simulink model "TIM_5_1_2"  (R2022b)
(part 2 of 4)

  Nex_1 (3) : M-S-Function  FunctionName=cisia_msfun  Parameters=Parameter1, Parameter2, Parameter3, resources, Parameter10, codeupdate, step_received, step_computed, dynamic_computed, step_sended, id_entity, id_project, id_type, name_type, color  mask(S-function:msfcn_unit_delay){Parameter1='Nex_1', Parameter2=1, Parameter3='ORO', resources=*** INPUT RESOURCES *** NUM_INPUTS 5 TLC_CONN (20) TLC_SERVICE (20) CYBER_FAULT (10) POWER (1) ROOM_QoS (1)  *** STATE VARIABLES *** NUM_VARIABLES 17 Operative_Level(NUMERIC)(1)(1) TLC_services(NUMERIC_ARRAY)(20)(0  0  0  0  0  0  0  0  0  0  0  0  0  0  0  0  0  0  0  0) Connection(NUMERIC_ARRAY)(20)(0  0  0  0  0  0  0  0  0  0  0  0  0  0  0  0  0  0  0  0) Dos_attack(NUMERIC)(1)(0) MITM_attack(NUMERIC)(1)(0) Virus_Attack(NUMERIC)(1)(0) Port_Scan_Attack(NUMERIC)(1)(0) Cyber_Fault(NUMERIC_ARRAY)(10)(0  0  0  0  0  0  0  0  0  0) BGP_hijacking(NUMERIC)(1)(0) Mechanical_Fault(NUMERIC)(1)(0) Conn_Fault(NUMERIC)(1)(0) BotNet_Attack(NUMERIC)(1)(0) Data_Corruption(NUMERIC)(1)(0) SW_Change(NUMERIC)(1)(0) Config_Change(NUMERIC)(1)(0) Port_Saturation(NUMERIC)(1)(0) TLC_revoke(NUMERIC_ARRAY)(20)(0  0  0  0  0  0  0  0  0  0  0  0  0  0  0  0  0  0  0  0)  *** OUTPUT RESOURCES *** NUM_OUTPUTS 4 TLC_CONN (20) TLC_SERVICE (20) CYBER_FAULT (10) SWITCHING_QoS (1), Parameter10=off, codeupdate=off, step_received=Connection=max(Connection_init,TLC_CONN);  TLC_services=max(TLC_services_init,TLC_SERVICE); TLC_services=mod(TLC_services,10); TLC_revoke=floor(TLC_SERVICE/10);  Cyber_Fault=max(CYBER_FAULT, transpose([Dos_attack   MITM_attack Virus_Attack Port_Scan_Attack  BGP_hijacking BotNet_Attack Data_Corruption SW_Change Config_Change Port_Saturation]));  Conn_Fault=max([Dos_attack  Mechanical_Fault  1-POWER 1-ROOM_QoS] );  Operative_Level=(1-Conn_Fault)*max(max(TLC_services),0.5)*(1-0.5*max(Cyber_Fault));, step_computed=, dynamic_computed=, step_sended=TLC_CONN=Connection*(1-Conn_Fault); TLC_SERVICE=TLC_services*(1-Conn_Fault)+10*TLC_revoke;  Cyber_Transmitted=min(Cyber_Fault, transpose([0 0 1 0 1 1 0 0 0 1])); CYBER_FAULT=Cyber_Transmitted*(1-Conn_Fault);   SWITCHING_QoS=Operative_Level;, id_entity=3, id_project=38, id_type=2, name_type=Nexus93180Switch, color=#0072BD}
      mask prompts: Parameter1 "entity name"; Parameter2 "sampling time"; Parameter3 "project"; resources "input resources and state variables"; Parameter10 "Bring state variables to output"; codeupdate "update code from mask"
      mask help: This is a level-2 MATLAB file S-function which demonstrates CISIA entity
      mask DialogControl Container1 Prompt: All parameters
      mask Display: image('Icons/Nexus93180Switch.png')
  Nex_2 (4) : M-S-Function  FunctionName=cisia_msfun  Parameters=Parameter1, Parameter2, Parameter3, resources, Parameter10, codeupdate, step_received, step_computed, dynamic_computed, step_sended, id_entity, id_project, id_type, name_type, color  mask(S-function:msfcn_unit_delay){Parameter1='Nex_2', Parameter2=1, Parameter3='ORO', resources=*** INPUT RESOURCES *** NUM_INPUTS 5 TLC_CONN (20) TLC_SERVICE (20) CYBER_FAULT (10) POWER (1) ROOM_QoS (1)  *** STATE VARIABLES *** NUM_VARIABLES 17 Operative_Level(NUMERIC)(1)(1) TLC_services(NUMERIC_ARRAY)(20)(0  0  0  0  0  0  0  0  0  0  0  0  0  0  0  0  0  0  0  0) Connection(NUMERIC_ARRAY)(20)(0  0  0  0  0  0  0  0  0  0  0  0  0  0  0  0  0  0  0  0) Dos_attack(NUMERIC)(1)(0) MITM_attack(NUMERIC)(1)(0) Virus_Attack(NUMERIC)(1)(0) Port_Scan_Attack(NUMERIC)(1)(0) Cyber_Fault(NUMERIC_ARRAY)(10)(0  0  0  0  0  0  0  0  0  0) BGP_hijacking(NUMERIC)(1)(0) Mechanical_Fault(NUMERIC)(1)(0) Conn_Fault(NUMERIC)(1)(0) BotNet_Attack(NUMERIC)(1)(0) Data_Corruption(NUMERIC)(1)(0) SW_Change(NUMERIC)(1)(0) Config_Change(NUMERIC)(1)(0) Port_Saturation(NUMERIC)(1)(0) TLC_revoke(NUMERIC_ARRAY)(20)(0  0  0  0  0  0  0  0  0  0  0  0  0  0  0  0  0  0  0  0)  *** OUTPUT RESOURCES *** NUM_OUTPUTS 4 TLC_CONN (20) TLC_SERVICE (20) CYBER_FAULT (10) SWITCHING_QoS (1), Parameter10=off, codeupdate=off, step_received=Connection=max(Connection_init,TLC_CONN);  TLC_services=max(TLC_services_init,TLC_SERVICE); TLC_services=mod(TLC_services,10); TLC_revoke=floor(TLC_SERVICE/10);  Cyber_Fault=max(CYBER_FAULT, transpose([Dos_attack   MITM_attack Virus_Attack Port_Scan_Attack  BGP_hijacking BotNet_Attack Data_Corruption SW_Change Config_Change Port_Saturation]));  Conn_Fault=max([Dos_attack  Mechanical_Fault  1-POWER 1-ROOM_QoS] );  Operative_Level=(1-Conn_Fault)*max(max(TLC_services),0.5)*(1-0.5*max(Cyber_Fault));, step_computed=, dynamic_computed=, step_sended=TLC_CONN=Connection*(1-Conn_Fault); TLC_SERVICE=TLC_services*(1-Conn_Fault)+10*TLC_revoke;  Cyber_Transmitted=min(Cyber_Fault, transpose([0 0 1 0 1 1 0 0 0 1])); CYBER_FAULT=Cyber_Transmitted*(1-Conn_Fault);   SWITCHING_QoS=Operative_Level;, id_entity=4, id_project=38, id_type=2, name_type=Nexus93180Switch, color=#0072BD}
      mask prompts: Parameter1 "entity name"; Parameter2 "sampling time"; Parameter3 "project"; resources "input resources and state variables"; Parameter10 "Bring state variables to output"; codeupdate "update code from mask"
      mask help: This is a level-2 MATLAB file S-function which demonstrates CISIA entity
      mask DialogControl Container1 Prompt: All parameters
      mask Display: image('Icons/Nexus93180Switch.png')
  ONU_3 (282) : M-S-Function  FunctionName=cisia_msfun  Parameters=Parameter1, Parameter2, Parameter3, resources, Parameter10, codeupdate, step_received, step_computed, dynamic_computed, step_sended, id_entity, id_project, id_type, name_type, color  mask(S-function:msfcn_unit_delay){Parameter1='ONU_3', Parameter2=1, Parameter3='ORO', resources=*** INPUT RESOURCES *** NUM_INPUTS 4 TLC_SERVICE (20) CYBER_FAULT (10) POWER (1) NGPON_CONN (20)  *** STATE VARIABLES *** NUM_VARIABLES 22 Operative_Level(NUMERIC)(1)(1) TLC_services(NUMERIC_ARRAY)(20)(0  0  0  0  0  0  0  0  0  0  0  0  0  0  0  0  0  0  0  0) Connection(NUMERIC_ARRAY)(20)(0  0  0  0  0  0  0  0  0  0  0  0  0  0  0  0  0  0  0  0) Dos_attack(NUMERIC)(1)(0) MITM_attack(NUMERIC)(1)(0) Virus_Attack(NUMERIC)(1)(0) Port_Scan_Attack(NUMERIC)(1)(0) Cyber_Fault(NUMERIC_ARRAY)(10)(0  0  0  0  0  0  0  0  0  0) MyConn(NUMERIC_ARRAY)(20)(0  0  0  0  0  0  0  0  0  0  0  0  0  0  0  0  0  0  0  0) BGP_hijacking(NUMERIC)(1)(0) Mechanical_Fault(NUMERIC)(1)(0) Conn_Fault(NUMERIC)(1)(0) Consumed_Services(NUMERIC_ARRAY)(20)(0  0  0  0  0  0  0  0  0  0  0  0  0  0  0  0  0  0  0  0) Service_Fault(NUMERIC)(1)(0) Redundancy_Fault(NUMERIC)(1)(0) BotNet_Attack(NUMERIC)(1)(0) Data_Corruption(NUMERIC)(1)(0) SW_Change(NUMERIC)(1)(0) Config_Change(NUMERIC)(1)(0) Port_Saturation(NUMERIC)(1)(0) My_Service(NUMERIC)(1)(0) TLC_revoke(NUMERIC_ARRAY)(20)(0  0  0  0  0  0  0  0  0  0  0  0  0  0  0  0  0  0  0  0)  *** OUTPUT RESOURCES *** NUM_OUTPUTS 3 TLC_SERVICE (20) CYBER_FAULT (10) NGPON_CONN (20), Parameter10=off, codeupdate=off, step_received=Connection=max(Connection_init,NGPON_CONN); TLC_services=max(TLC_services_init,TLC_SERVICE); TLC_services=mod(TLC_services,10); TLC_revoke=floor(TLC_SERVICE/10);  Cyber_Fault=max(CYBER_FAULT, transpose([Dos_attack   MITM_attack Virus_Attack Port_Scan_Attack  BGP_hijacking BotNet_Attack Data_Corruption SW_Change Config_Change Port_Saturation]));  Conn_Fault=max([Dos_attack  Mechanical_Fault  1-POWER] );  Service_Fault=max(abs(Consumed_Services.*TLC_services-Consumed_Services)); Redundancy_Fault=max(abs(Consumed_Services.*NGPON_CONN-Consumed_Services));  Operative_Level=(1-Conn_Fault)*(1-0.5*max(Cyber_Fault))*(1-Service_Fault)*max(max(NGPON_CONN),0.5);  %Operative_Level=(1-Conn_Fault)*max(max(TLC_services),0.5)*((2*(1-Service_Fault)+(1-Redundancy_Fault))/3); % Il servizio utilizzato %My_Service=max([(1-Service_Fault) (1-Redundancy_Fault)/2]); %Operative_Level=(1-Conn_Fault);, step_computed=, dynamic_computed=, step_sended=TLC_SERVICE=TLC_services*(1-Conn_Fault)+10*TLC_revoke; NGPON_CONN=Connection*(1-Conn_Fault);  Cyber_Transmitted=min(Cyber_Fault, transpose([0 0 1 0 1 1 0 0 0 1])); CYBER_FAULT=Cyber_Transmitted*(1-Conn_Fault);, id_entity=282, id_project=38, id_type=12, name_type=ONU, color=#90DB5A}
      mask prompts: Parameter1 "entity name"; Parameter2 "sampling time"; Parameter3 "project"; resources "input resources and state variables"; Parameter10 "Bring state variables to output"; codeupdate "update code from mask"
      mask help: This is a level-2 MATLAB file S-function which demonstrates CISIA entity
      mask DialogControl Container1 Prompt: All parameters
      mask Display: disp('ONU')
  Operating_1 (177) : M-S-Function  FunctionName=cisia_msfun  Parameters=Parameter1, Parameter2, Parameter3, resources, Parameter10, codeupdate, step_received, step_computed, dynamic_computed, step_sended, id_entity, id_project, id_type, name_type, color  mask(S-function:msfcn_unit_delay){Parameter1='Operating_1', Parameter2=1, Parameter3='ORO', resources=*** INPUT RESOURCES *** NUM_INPUTS 8 TLC_CONN (20) TLC_SERVICE (20) CYBER_FAULT (10) POWER (1) WATER (1) AIR (1) MOBILE_QoS (1) OXYGEN (1)  *** STATE VARIABLES *** NUM_VARIABLES 17 Operative_Level(NUMERIC)(1)(1) TLC_services(NUMERIC_ARRAY)(20)(0  0  0  0  0  0  0  0  0  0  0  0  0  0  0  0  0  0  0  0) Connection(NUMERIC_ARRAY)(20)(0  0  0  0  0  0  0  0  0  0  0  0  0  0  0  0  0  0  0  0) Mechanical_Fault(NUMERIC)(1)(0) Power_Fault(NUMERIC)(1)(0) Fire_Fault(NUMERIC)(1)(0) Conn_Fault(NUMERIC)(1)(0) Consumed_Services(NUMERIC_ARRAY)(20)(0  0  0  0  1  0  0  0  1  0  0  0  0  0  0  0  0  0  0  0) Service_Fault(NUMERIC)(1)(0) Redundancy_Fault(NUMERIC)(1)(0) Water_Fault(NUMERIC)(1)(0) Air_Fault(NUMERIC)(1)(0) Physical_Fault(NUMERIC)(1)(0) TLC_revoke(NUMERIC_ARRAY)(20)(0  0  0  0  0  0  0  0  0  0  0  0  0  0  0  0  0  0  0  0) Alternative_Services(NUMERIC_ARRAY)(20)(0  0  0  0  0  0  0  0  0  0  0  0  0  0  0  0  0  0  0  0) Alt_Serv_Fault(NUMERIC)(1)(0) Alt_Rout_Fault(NUMERIC)(1)(0)  *** OUTPUT RESOURCES *** NUM_OUTPUTS 3 MEDICAL_ROOM_QoS (1) ALT_ROUTING (1) ALT_SERVICES (1), Parameter10=off, codeupdate=off, step_received=Connection=max(Connection_init,TLC_CONN); TLC_services=max(TLC_services_init,TLC_SERVICE); TLC_services=mod(TLC_services,10); TLC_revoke=floor(TLC_SERVICE/10);  Conn_Fault=max([Power_Fault 1-POWER 1-MOBILE_QoS]);  Water_Fault=1-WATER; Air_Fault=1-AIR; Physical_Fault=max([Water_Fault Air_Fault 1-OXYGEN]);  Alt_Serv_Fault=max(abs(Alternative_Services.*TLC_CONN-Alternative_Services));  Alt_Rout_Fault=max(abs(Consumed_Services.*TLC_CONN-Consumed_Services));   Service_Fault=max(abs(Consumed_Services.*TLC_services-Consumed_Services)); Redundancy_Fault=max(abs(Consumed_Services.*TLC_CONN-Consumed_Services));  Operative_Level=(1-Conn_Fault)*(1-0.5*Physical_Fault)*(1-0.5*Service_Fault);, step_computed=, dynamic_computed=, step_sended=MEDICAL_ROOM_QoS=Operative_Level;  ALT_SERVICES=1-Alt_Serv_Fault; ALT_ROUTING=1-Alt_Rout_Fault;, id_entity=177, id_project=38, id_type=25, name_type=Medical_Room, color=#00FFFF}
      mask prompts: Parameter1 "entity name"; Parameter2 "sampling time"; Parameter3 "project"; resources "input resources and state variables"; Parameter10 "Bring state variables to output"; codeupdate "update code from mask"
      mask help: This is a level-2 MATLAB file S-function which demonstrates CISIA entity
      mask DialogControl Container1 Prompt: All parameters
      mask Display: disp('Medical_Room')
  Operating_2 (178) : M-S-Function  FunctionName=cisia_msfun  Parameters=Parameter1, Parameter2, Parameter3, resources, Parameter10, codeupdate, step_received, step_computed, dynamic_computed, step_sended, id_entity, id_project, id_type, name_type, color  mask(S-function:msfcn_unit_delay){Parameter1='Operating_2', Parameter2=1, Parameter3='ORO', resources=*** INPUT RESOURCES *** NUM_INPUTS 8 TLC_CONN (20) TLC_SERVICE (20) CYBER_FAULT (10) POWER (1) WATER (1) AIR (1) MOBILE_QoS (1) OXYGEN (1)  *** STATE VARIABLES *** NUM_VARIABLES 17 Operative_Level(NUMERIC)(1)(1) TLC_services(NUMERIC_ARRAY)(20)(0  0  0  0  0  0  0  0  0  0  0  0  0  0  0  0  0  0  0  0) Connection(NUMERIC_ARRAY)(20)(0  0  0  0  0  0  0  0  0  0  0  0  0  0  0  0  0  0  0  0) Mechanical_Fault(NUMERIC)(1)(0) Power_Fault(NUMERIC)(1)(0) Fire_Fault(NUMERIC)(1)(0) Conn_Fault(NUMERIC)(1)(0) Consumed_Services(NUMERIC_ARRAY)(20)(0  0  0  0  1  0  0  0  1  0  0  0  0  0  0  0  0  0  0  0) Service_Fault(NUMERIC)(1)(0) Redundancy_Fault(NUMERIC)(1)(0) Water_Fault(NUMERIC)(1)(0) Air_Fault(NUMERIC)(1)(0) Physical_Fault(NUMERIC)(1)(0) TLC_revoke(NUMERIC_ARRAY)(20)(0  0  0  0  0  0  0  0  0  0  0  0  0  0  0  0  0  0  0  0) Alternative_Services(NUMERIC_ARRAY)(20)(0  0  0  0  0  0  0  0  0  0  0  0  0  0  0  0  0  0  0  0) Alt_Serv_Fault(NUMERIC)(1)(0) Alt_Rout_Fault(NUMERIC)(1)(0)  *** OUTPUT RESOURCES *** NUM_OUTPUTS 3 MEDICAL_ROOM_QoS (1) ALT_ROUTING (1) ALT_SERVICES (1), Parameter10=off, codeupdate=off, step_received=Connection=max(Connection_init,TLC_CONN); TLC_services=max(TLC_services_init,TLC_SERVICE); TLC_services=mod(TLC_services,10); TLC_revoke=floor(TLC_SERVICE/10);  Conn_Fault=max([Power_Fault 1-POWER 1-MOBILE_QoS]);  Water_Fault=1-WATER; Air_Fault=1-AIR; Physical_Fault=max([Water_Fault Air_Fault 1-OXYGEN]);  Alt_Serv_Fault=max(abs(Alternative_Services.*TLC_CONN-Alternative_Services));  Alt_Rout_Fault=max(abs(Consumed_Services.*TLC_CONN-Consumed_Services));   Service_Fault=max(abs(Consumed_Services.*TLC_services-Consumed_Services)); Redundancy_Fault=max(abs(Consumed_Services.*TLC_CONN-Consumed_Services));  Operative_Level=(1-Conn_Fault)*(1-0.5*Physical_Fault)*(1-0.5*Service_Fault);, step_computed=, dynamic_computed=, step_sended=MEDICAL_ROOM_QoS=Operative_Level;  ALT_SERVICES=1-Alt_Serv_Fault; ALT_ROUTING=1-Alt_Rout_Fault;, id_entity=178, id_project=38, id_type=25, name_type=Medical_Room, color=#00FFFF}
      mask prompts: Parameter1 "entity name"; Parameter2 "sampling time"; Parameter3 "project"; resources "input resources and state variables"; Parameter10 "Bring state variables to output"; codeupdate "update code from mask"
      mask help: This is a level-2 MATLAB file S-function which demonstrates CISIA entity
      mask DialogControl Container1 Prompt: All parameters
      mask Display: disp('Medical_Room')
  Oxygen_Duct_1 (263) : M-S-Function  FunctionName=cisia_msfun  Parameters=Parameter1, Parameter2, Parameter3, resources, Parameter10, codeupdate, step_received, step_computed, dynamic_computed, step_sended, id_entity, id_project, id_type, name_type, color  mask(S-function:msfcn_unit_delay){Parameter1='Oxygen_Duct_1', Parameter2=1, Parameter3='ORO', resources=*** INPUT RESOURCES *** NUM_INPUTS 1 OXYGEN (1)  *** STATE VARIABLES *** NUM_VARIABLES 2 Operative_Level(NUMERIC)(1)(1) Mechanical_Fault(NUMERIC)(1)(0)  *** OUTPUT RESOURCES *** NUM_OUTPUTS 1 OXYGEN (1), Parameter10=off, codeupdate=off, step_received=Operative_Level=(1-Mechanical_Fault)*(1-0.5*(1-OXYGEN));, step_computed=, dynamic_computed=, step_sended=OXYGEN=Operative_Level;, id_entity=263, id_project=38, id_type=57, name_type=OXYGEN_Duct, color=#E85151}
      mask prompts: Parameter1 "entity name"; Parameter2 "sampling time"; Parameter3 "project"; resources "input resources and state variables"; Parameter10 "Bring state variables to output"; codeupdate "update code from mask"
      mask help: This is a level-2 MATLAB file S-function which demonstrates CISIA entity
      mask DialogControl Container1 Prompt: All parameters
      mask Display: disp('OXYGEN_Duct')
  Oxygen_Duct_2 (264) : M-S-Function  FunctionName=cisia_msfun  Parameters=Parameter1, Parameter2, Parameter3, resources, Parameter10, codeupdate, step_received, step_computed, dynamic_computed, step_sended, id_entity, id_project, id_type, name_type, color  mask(S-function:msfcn_unit_delay){Parameter1='Oxygen_Duct_2', Parameter2=1, Parameter3='ORO', resources=*** INPUT RESOURCES *** NUM_INPUTS 1 OXYGEN (1)  *** STATE VARIABLES *** NUM_VARIABLES 2 Operative_Level(NUMERIC)(1)(1) Mechanical_Fault(NUMERIC)(1)(0)  *** OUTPUT RESOURCES *** NUM_OUTPUTS 1 OXYGEN (1), Parameter10=off, codeupdate=off, step_received=Operative_Level=(1-Mechanical_Fault)*(1-0.5*(1-OXYGEN));, step_computed=, dynamic_computed=, step_sended=OXYGEN=Operative_Level;, id_entity=264, id_project=38, id_type=57, name_type=OXYGEN_Duct, color=#E85151}
      mask prompts: Parameter1 "entity name"; Parameter2 "sampling time"; Parameter3 "project"; resources "input resources and state variables"; Parameter10 "Bring state variables to output"; codeupdate "update code from mask"
      mask help: This is a level-2 MATLAB file S-function which demonstrates CISIA entity
      mask DialogControl Container1 Prompt: All parameters
      mask Display: disp('OXYGEN_Duct')
  Oxygen_Duct_3 (265) : M-S-Function  FunctionName=cisia_msfun  Parameters=Parameter1, Parameter2, Parameter3, resources, Parameter10, codeupdate, step_received, step_computed, dynamic_computed, step_sended, id_entity, id_project, id_type, name_type, color  mask(S-function:msfcn_unit_delay){Parameter1='Oxygen_Duct_3', Parameter2=1, Parameter3='ORO', resources=*** INPUT RESOURCES *** NUM_INPUTS 1 OXYGEN (1)  *** STATE VARIABLES *** NUM_VARIABLES 2 Operative_Level(NUMERIC)(1)(1) Mechanical_Fault(NUMERIC)(1)(0)  *** OUTPUT RESOURCES *** NUM_OUTPUTS 1 OXYGEN (1), Parameter10=off, codeupdate=off, step_received=Operative_Level=(1-Mechanical_Fault)*(1-0.5*(1-OXYGEN));, step_computed=, dynamic_computed=, step_sended=OXYGEN=Operative_Level;, id_entity=265, id_project=38, id_type=57, name_type=OXYGEN_Duct, color=#E85151}
      mask prompts: Parameter1 "entity name"; Parameter2 "sampling time"; Parameter3 "project"; resources "input resources and state variables"; Parameter10 "Bring state variables to output"; codeupdate "update code from mask"
      mask help: This is a level-2 MATLAB file S-function which demonstrates CISIA entity
      mask DialogControl Container1 Prompt: All parameters
      mask Display: disp('OXYGEN_Duct')
  Oxygen_Duct_4 (266) : M-S-Function  FunctionName=cisia_msfun  Parameters=Parameter1, Parameter2, Parameter3, resources, Parameter10, codeupdate, step_received, step_computed, dynamic_computed, step_sended, id_entity, id_project, id_type, name_type, color  mask(S-function:msfcn_unit_delay){Parameter1='Oxygen_Duct_4', Parameter2=1, Parameter3='ORO', resources=*** INPUT RESOURCES *** NUM_INPUTS 1 OXYGEN (1)  *** STATE VARIABLES *** NUM_VARIABLES 2 Operative_Level(NUMERIC)(1)(1) Mechanical_Fault(NUMERIC)(1)(0)  *** OUTPUT RESOURCES *** NUM_OUTPUTS 1 OXYGEN (1), Parameter10=off, codeupdate=off, step_received=Operative_Level=(1-Mechanical_Fault)*(1-0.5*(1-OXYGEN));, step_computed=, dynamic_computed=, step_sended=OXYGEN=Operative_Level;, id_entity=266, id_project=38, id_type=57, name_type=OXYGEN_Duct, color=#E85151}
      mask prompts: Parameter1 "entity name"; Parameter2 "sampling time"; Parameter3 "project"; resources "input resources and state variables"; Parameter10 "Bring state variables to output"; codeupdate "update code from mask"
      mask help: This is a level-2 MATLAB file S-function which demonstrates CISIA entity
      mask DialogControl Container1 Prompt: All parameters
      mask Display: disp('OXYGEN_Duct')
  Oxygen_Duct_5 (267) : M-S-Function  FunctionName=cisia_msfun  Parameters=Parameter1, Parameter2, Parameter3, resources, Parameter10, codeupdate, step_received, step_computed, dynamic_computed, step_sended, id_entity, id_project, id_type, name_type, color  mask(S-function:msfcn_unit_delay){Parameter1='Oxygen_Duct_5', Parameter2=1, Parameter3='ORO', resources=*** INPUT RESOURCES *** NUM_INPUTS 1 OXYGEN (1)  *** STATE VARIABLES *** NUM_VARIABLES 2 Operative_Level(NUMERIC)(1)(1) Mechanical_Fault(NUMERIC)(1)(0)  *** OUTPUT RESOURCES *** NUM_OUTPUTS 1 OXYGEN (1), Parameter10=off, codeupdate=off, step_received=Operative_Level=(1-Mechanical_Fault)*(1-0.5*(1-OXYGEN));, step_computed=, dynamic_computed=, step_sended=OXYGEN=Operative_Level;, id_entity=267, id_project=38, id_type=57, name_type=OXYGEN_Duct, color=#E85151}
      mask prompts: Parameter1 "entity name"; Parameter2 "sampling time"; Parameter3 "project"; resources "input resources and state variables"; Parameter10 "Bring state variables to output"; codeupdate "update code from mask"
      mask help: This is a level-2 MATLAB file S-function which demonstrates CISIA entity
      mask DialogControl Container1 Prompt: All parameters
      mask Display: disp('OXYGEN_Duct')
  Oxygen_Duct_6 (268) : M-S-Function  FunctionName=cisia_msfun  Parameters=Parameter1, Parameter2, Parameter3, resources, Parameter10, codeupdate, step_received, step_computed, dynamic_computed, step_sended, id_entity, id_project, id_type, name_type, color  mask(S-function:msfcn_unit_delay){Parameter1='Oxygen_Duct_6', Parameter2=1, Parameter3='ORO', resources=*** INPUT RESOURCES *** NUM_INPUTS 1 OXYGEN (1)  *** STATE VARIABLES *** NUM_VARIABLES 2 Operative_Level(NUMERIC)(1)(1) Mechanical_Fault(NUMERIC)(1)(0)  *** OUTPUT RESOURCES *** NUM_OUTPUTS 1 OXYGEN (1), Parameter10=off, codeupdate=off, step_received=Operative_Level=(1-Mechanical_Fault)*(1-0.5*(1-OXYGEN));, step_computed=, dynamic_computed=, step_sended=OXYGEN=Operative_Level;, id_entity=268, id_project=38, id_type=57, name_type=OXYGEN_Duct, color=#E85151}
      mask prompts: Parameter1 "entity name"; Parameter2 "sampling time"; Parameter3 "project"; resources "input resources and state variables"; Parameter10 "Bring state variables to output"; codeupdate "update code from mask"
      mask help: This is a level-2 MATLAB file S-function which demonstrates CISIA entity
      mask DialogControl Container1 Prompt: All parameters
      mask Display: disp('OXYGEN_Duct')
  Oxygen_Duct_7 (269) : M-S-Function  FunctionName=cisia_msfun  Parameters=Parameter1, Parameter2, Parameter3, resources, Parameter10, codeupdate, step_received, step_computed, dynamic_computed, step_sended, id_entity, id_project, id_type, name_type, color  mask(S-function:msfcn_unit_delay){Parameter1='Oxygen_Duct_7', Parameter2=1, Parameter3='ORO', resources=*** INPUT RESOURCES *** NUM_INPUTS 1 OXYGEN (1)  *** STATE VARIABLES *** NUM_VARIABLES 2 Operative_Level(NUMERIC)(1)(1) Mechanical_Fault(NUMERIC)(1)(0)  *** OUTPUT RESOURCES *** NUM_OUTPUTS 1 OXYGEN (1), Parameter10=off, codeupdate=off, step_received=Operative_Level=(1-Mechanical_Fault)*(1-0.5*(1-OXYGEN));, step_computed=, dynamic_computed=, step_sended=OXYGEN=Operative_Level;, id_entity=269, id_project=38, id_type=57, name_type=OXYGEN_Duct, color=#E85151}
      mask prompts: Parameter1 "entity name"; Parameter2 "sampling time"; Parameter3 "project"; resources "input resources and state variables"; Parameter10 "Bring state variables to output"; codeupdate "update code from mask"
      mask help: This is a level-2 MATLAB file S-function which demonstrates CISIA entity
      mask DialogControl Container1 Prompt: All parameters
      mask Display: disp('OXYGEN_Duct')
  Oxygen_Duct_8 (270) : M-S-Function  FunctionName=cisia_msfun  Parameters=Parameter1, Parameter2, Parameter3, resources, Parameter10, codeupdate, step_received, step_computed, dynamic_computed, step_sended, id_entity, id_project, id_type, name_type, color  mask(S-function:msfcn_unit_delay){Parameter1='Oxygen_Duct_8', Parameter2=1, Parameter3='ORO', resources=*** INPUT RESOURCES *** NUM_INPUTS 1 OXYGEN (1)  *** STATE VARIABLES *** NUM_VARIABLES 2 Operative_Level(NUMERIC)(1)(1) Mechanical_Fault(NUMERIC)(1)(0)  *** OUTPUT RESOURCES *** NUM_OUTPUTS 1 OXYGEN (1), Parameter10=off, codeupdate=off, step_received=Operative_Level=(1-Mechanical_Fault)*(1-0.5*(1-OXYGEN));, step_computed=, dynamic_computed=, step_sended=OXYGEN=Operative_Level;, id_entity=270, id_project=38, id_type=57, name_type=OXYGEN_Duct, color=#E85151}
      mask prompts: Parameter1 "entity name"; Parameter2 "sampling time"; Parameter3 "project"; resources "input resources and state variables"; Parameter10 "Bring state variables to output"; codeupdate "update code from mask"
      mask help: This is a level-2 MATLAB file S-function which demonstrates CISIA entity
      mask DialogControl Container1 Prompt: All parameters
      mask Display: disp('OXYGEN_Duct')
  Oxygen_Pump (251) : M-S-Function  FunctionName=cisia_msfun  Parameters=Parameter1, Parameter2, Parameter3, resources, Parameter10, codeupdate, step_received, step_computed, dynamic_computed, step_sended, id_entity, id_project, id_type, name_type, color  mask(S-function:msfcn_unit_delay){Parameter1='Oxygen_Pump', Parameter2=1, Parameter3='ORO', resources=*** INPUT RESOURCES *** NUM_INPUTS 1 POWER (1)  *** STATE VARIABLES *** NUM_VARIABLES 3 Operative_Level(NUMERIC)(1)(1) Mechanical_Fault(NUMERIC)(1)(0) Power_Fault(NUMERIC)(1)(0)  *** OUTPUT RESOURCES *** NUM_OUTPUTS 1 OXYGEN (1), Parameter10=off, codeupdate=off, step_received=Power_Fault=(1-POWER); Operative_Level=(1-Mechanical_Fault)*(1-0.5*Power_Fault);, step_computed=, dynamic_computed=, step_sended=OXYGEN=Operative_Level;, id_entity=251, id_project=38, id_type=56, name_type=OXYGEN_Element, color=#A11326}
      mask prompts: Parameter1 "entity name"; Parameter2 "sampling time"; Parameter3 "project"; resources "input resources and state variables"; Parameter10 "Bring state variables to output"; codeupdate "update code from mask"
      mask help: This is a level-2 MATLAB file S-function which demonstrates CISIA entity
      mask DialogControl Container1 Prompt: All parameters
      mask Display: disp('OXYGEN_Element')
  Pipe_1 (120) : M-S-Function  FunctionName=cisia_msfun  Parameters=Parameter1, Parameter2, Parameter3, resources, Parameter10, codeupdate, step_received, step_computed, dynamic_computed, step_sended, id_entity, id_project, id_type, name_type, color  mask(S-function:msfcn_unit_delay){Parameter1='Pipe_1', Parameter2=1, Parameter3='ORO', resources=*** INPUT RESOURCES *** NUM_INPUTS 1 WATER (1)  *** STATE VARIABLES *** NUM_VARIABLES 3 Operative_Level(NUMERIC)(1)(1) Mechanical_Fault(NUMERIC)(1)(0) Water_Fault(NUMERIC)(1)(0)  *** OUTPUT RESOURCES *** NUM_OUTPUTS 2 WATER (1) PIPE_QoS (1), Parameter10=off, codeupdate=off, step_received=Water_Fault= 1- WATER; Operative_Level=(1-Mechanical_Fault)*(1-0.5*Water_Fault);, step_computed=, dynamic_computed=, step_sended=WATER=Operative_Level; PIPE_QoS=Operative_Level;, id_entity=120, id_project=38, id_type=32, name_type=Pipe, color=#78C6FA}
      mask prompts: Parameter1 "entity name"; Parameter2 "sampling time"; Parameter3 "project"; resources "input resources and state variables"; Parameter10 "Bring state variables to output"; codeupdate "update code from mask"
      mask help: This is a level-2 MATLAB file S-function which demonstrates CISIA entity
      mask DialogControl Container1 Prompt: All parameters
      mask Display: image('Icons/Pipe.png')
  Pipe_Medical1 (128) : M-S-Function  FunctionName=cisia_msfun  Parameters=Parameter1, Parameter2, Parameter3, resources, Parameter10, codeupdate, step_received, step_computed, dynamic_computed, step_sended, id_entity, id_project, id_type, name_type, color  mask(S-function:msfcn_unit_delay){Parameter1='Pipe_Medical1', Parameter2=1, Parameter3='ORO', resources=*** INPUT RESOURCES *** NUM_INPUTS 1 WATER (1)  *** STATE VARIABLES *** NUM_VARIABLES 3 Operative_Level(NUMERIC)(1)(1) Mechanical_Fault(NUMERIC)(1)(0) Water_Fault(NUMERIC)(1)(0)  *** OUTPUT RESOURCES *** NUM_OUTPUTS 2 WATER (1) PIPE_QoS (1), Parameter10=off, codeupdate=off, step_received=Water_Fault= 1- WATER; Operative_Level=(1-Mechanical_Fault)*(1-0.5*Water_Fault);, step_computed=, dynamic_computed=, step_sended=WATER=Operative_Level; PIPE_QoS=Operative_Level;, id_entity=128, id_project=38, id_type=32, name_type=Pipe, color=#78C6FA}
      mask prompts: Parameter1 "entity name"; Parameter2 "sampling time"; Parameter3 "project"; resources "input resources and state variables"; Parameter10 "Bring state variables to output"; codeupdate "update code from mask"
      mask help: This is a level-2 MATLAB file S-function which demonstrates CISIA entity
      mask DialogControl Container1 Prompt: All parameters
      mask Display: image('Icons/Pipe.png')
  Pipe_Medical2 (129) : M-S-Function  FunctionName=cisia_msfun  Parameters=Parameter1, Parameter2, Parameter3, resources, Parameter10, codeupdate, step_received, step_computed, dynamic_computed, step_sended, id_entity, id_project, id_type, name_type, color  mask(S-function:msfcn_unit_delay){Parameter1='Pipe_Medical2', Parameter2=1, Parameter3='ORO', resources=*** INPUT RESOURCES *** NUM_INPUTS 1 WATER (1)  *** STATE VARIABLES *** NUM_VARIABLES 3 Operative_Level(NUMERIC)(1)(1) Mechanical_Fault(NUMERIC)(1)(0) Water_Fault(NUMERIC)(1)(0)  *** OUTPUT RESOURCES *** NUM_OUTPUTS 2 WATER (1) PIPE_QoS (1), Parameter10=off, codeupdate=off, step_received=Water_Fault= 1- WATER; Operative_Level=(1-Mechanical_Fault)*(1-0.5*Water_Fault);, step_computed=, dynamic_computed=, step_sended=WATER=Operative_Level; PIPE_QoS=Operative_Level;, id_entity=129, id_project=38, id_type=32, name_type=Pipe, color=#78C6FA}
      mask prompts: Parameter1 "entity name"; Parameter2 "sampling time"; Parameter3 "project"; resources "input resources and state variables"; Parameter10 "Bring state variables to output"; codeupdate "update code from mask"
      mask help: This is a level-2 MATLAB file S-function which demonstrates CISIA entity
      mask DialogControl Container1 Prompt: All parameters
      mask Display: image('Icons/Pipe.png')
  Pipe_Medical3 (130) : M-S-Function  FunctionName=cisia_msfun  Parameters=Parameter1, Parameter2, Parameter3, resources, Parameter10, codeupdate, step_received, step_computed, dynamic_computed, step_sended, id_entity, id_project, id_type, name_type, color  mask(S-function:msfcn_unit_delay){Parameter1='Pipe_Medical3', Parameter2=1, Parameter3='ORO', resources=*** INPUT RESOURCES *** NUM_INPUTS 1 WATER (1)  *** STATE VARIABLES *** NUM_VARIABLES 3 Operative_Level(NUMERIC)(1)(1) Mechanical_Fault(NUMERIC)(1)(0) Water_Fault(NUMERIC)(1)(0)  *** OUTPUT RESOURCES *** NUM_OUTPUTS 2 WATER (1) PIPE_QoS (1), Parameter10=off, codeupdate=off, step_received=Water_Fault= 1- WATER; Operative_Level=(1-Mechanical_Fault)*(1-0.5*Water_Fault);, step_computed=, dynamic_computed=, step_sended=WATER=Operative_Level; PIPE_QoS=Operative_Level;, id_entity=130, id_project=38, id_type=32, name_type=Pipe, color=#78C6FA}
      mask prompts: Parameter1 "entity name"; Parameter2 "sampling time"; Parameter3 "project"; resources "input resources and state variables"; Parameter10 "Bring state variables to output"; codeupdate "update code from mask"
      mask help: This is a level-2 MATLAB file S-function which demonstrates CISIA entity
      mask DialogControl Container1 Prompt: All parameters
      mask Display: image('Icons/Pipe.png')
  Pipe_Medical4 (131) : M-S-Function  FunctionName=cisia_msfun  Parameters=Parameter1, Parameter2, Parameter3, resources, Parameter10, codeupdate, step_received, step_computed, dynamic_computed, step_sended, id_entity, id_project, id_type, name_type, color  mask(S-function:msfcn_unit_delay){Parameter1='Pipe_Medical4', Parameter2=1, Parameter3='ORO', resources=*** INPUT RESOURCES *** NUM_INPUTS 1 WATER (1)  *** STATE VARIABLES *** NUM_VARIABLES 3 Operative_Level(NUMERIC)(1)(1) Mechanical_Fault(NUMERIC)(1)(0) Water_Fault(NUMERIC)(1)(0)  *** OUTPUT RESOURCES *** NUM_OUTPUTS 2 WATER (1) PIPE_QoS (1), Parameter10=off, codeupdate=off, step_received=Water_Fault= 1- WATER; Operative_Level=(1-Mechanical_Fault)*(1-0.5*Water_Fault);, step_computed=, dynamic_computed=, step_sended=WATER=Operative_Level; PIPE_QoS=Operative_Level;, id_entity=131, id_project=38, id_type=32, name_type=Pipe, color=#78C6FA}
      mask prompts: Parameter1 "entity name"; Parameter2 "sampling time"; Parameter3 "project"; resources "input resources and state variables"; Parameter10 "Bring state variables to output"; codeupdate "update code from mask"
      mask help: This is a level-2 MATLAB file S-function which demonstrates CISIA entity
      mask DialogControl Container1 Prompt: All parameters
      mask Display: image('Icons/Pipe.png')
  Pipe_Medical5 (132) : M-S-Function  FunctionName=cisia_msfun  Parameters=Parameter1, Parameter2, Parameter3, resources, Parameter10, codeupdate, step_received, step_computed, dynamic_computed, step_sended, id_entity, id_project, id_type, name_type, color  mask(S-function:msfcn_unit_delay){Parameter1='Pipe_Medical5', Parameter2=1, Parameter3='ORO', resources=*** INPUT RESOURCES *** NUM_INPUTS 1 WATER (1)  *** STATE VARIABLES *** NUM_VARIABLES 3 Operative_Level(NUMERIC)(1)(1) Mechanical_Fault(NUMERIC)(1)(0) Water_Fault(NUMERIC)(1)(0)  *** OUTPUT RESOURCES *** NUM_OUTPUTS 2 WATER (1) PIPE_QoS (1), Parameter10=off, codeupdate=off, step_received=Water_Fault= 1- WATER; Operative_Level=(1-Mechanical_Fault)*(1-0.5*Water_Fault);, step_computed=, dynamic_computed=, step_sended=WATER=Operative_Level; PIPE_QoS=Operative_Level;, id_entity=132, id_project=38, id_type=32, name_type=Pipe, color=#78C6FA}
      mask prompts: Parameter1 "entity name"; Parameter2 "sampling time"; Parameter3 "project"; resources "input resources and state variables"; Parameter10 "Bring state variables to output"; codeupdate "update code from mask"
      mask help: This is a level-2 MATLAB file S-function which demonstrates CISIA entity
      mask DialogControl Container1 Prompt: All parameters
      mask Display: image('Icons/Pipe.png')
  Pipe_Medical6 (133) : M-S-Function  FunctionName=cisia_msfun  Parameters=Parameter1, Parameter2, Parameter3, resources, Parameter10, codeupdate, step_received, step_computed, dynamic_computed, step_sended, id_entity, id_project, id_type, name_type, color  mask(S-function:msfcn_unit_delay){Parameter1='Pipe_Medical6', Parameter2=1, Parameter3='ORO', resources=*** INPUT RESOURCES *** NUM_INPUTS 1 WATER (1)  *** STATE VARIABLES *** NUM_VARIABLES 3 Operative_Level(NUMERIC)(1)(1) Mechanical_Fault(NUMERIC)(1)(0) Water_Fault(NUMERIC)(1)(0)  *** OUTPUT RESOURCES *** NUM_OUTPUTS 2 WATER (1) PIPE_QoS (1), Parameter10=off, codeupdate=off, step_received=Water_Fault= 1- WATER; Operative_Level=(1-Mechanical_Fault)*(1-0.5*Water_Fault);, step_computed=, dynamic_computed=, step_sended=WATER=Operative_Level; PIPE_QoS=Operative_Level;, id_entity=133, id_project=38, id_type=32, name_type=Pipe, color=#78C6FA}
      mask prompts: Parameter1 "entity name"; Parameter2 "sampling time"; Parameter3 "project"; resources "input resources and state variables"; Parameter10 "Bring state variables to output"; codeupdate "update code from mask"
      mask help: This is a level-2 MATLAB file S-function which demonstrates CISIA entity
      mask DialogControl Container1 Prompt: All parameters
      mask Display: image('Icons/Pipe.png')
  Pipe_Oper1 (134) : M-S-Function  FunctionName=cisia_msfun  Parameters=Parameter1, Parameter2, Parameter3, resources, Parameter10, codeupdate, step_received, step_computed, dynamic_computed, step_sended, id_entity, id_project, id_type, name_type, color  mask(S-function:msfcn_unit_delay){Parameter1='Pipe_Oper1', Parameter2=1, Parameter3='ORO', resources=*** INPUT RESOURCES *** NUM_INPUTS 1 WATER (1)  *** STATE VARIABLES *** NUM_VARIABLES 3 Operative_Level(NUMERIC)(1)(1) Mechanical_Fault(NUMERIC)(1)(0) Water_Fault(NUMERIC)(1)(0)  *** OUTPUT RESOURCES *** NUM_OUTPUTS 2 WATER (1) PIPE_QoS (1), Parameter10=off, codeupdate=off, step_received=Water_Fault= 1- WATER; Operative_Level=(1-Mechanical_Fault)*(1-0.5*Water_Fault);, step_computed=, dynamic_computed=, step_sended=WATER=Operative_Level; PIPE_QoS=Operative_Level;, id_entity=134, id_project=38, id_type=32, name_type=Pipe, color=#78C6FA}
      mask prompts: Parameter1 "entity name"; Parameter2 "sampling time"; Parameter3 "project"; resources "input resources and state variables"; Parameter10 "Bring state variables to output"; codeupdate "update code from mask"
      mask help: This is a level-2 MATLAB file S-function which demonstrates CISIA entity
      mask DialogControl Container1 Prompt: All parameters
      mask Display: image('Icons/Pipe.png')
  Pipe_Oper2 (135) : M-S-Function  FunctionName=cisia_msfun  Parameters=Parameter1, Parameter2, Parameter3, resources, Parameter10, codeupdate, step_received, step_computed, dynamic_computed, step_sended, id_entity, id_project, id_type, name_type, color  mask(S-function:msfcn_unit_delay){Parameter1='Pipe_Oper2', Parameter2=1, Parameter3='ORO', resources=*** INPUT RESOURCES *** NUM_INPUTS 1 WATER (1)  *** STATE VARIABLES *** NUM_VARIABLES 3 Operative_Level(NUMERIC)(1)(1) Mechanical_Fault(NUMERIC)(1)(0) Water_Fault(NUMERIC)(1)(0)  *** OUTPUT RESOURCES *** NUM_OUTPUTS 2 WATER (1) PIPE_QoS (1), Parameter10=off, codeupdate=off, step_received=Water_Fault= 1- WATER; Operative_Level=(1-Mechanical_Fault)*(1-0.5*Water_Fault);, step_computed=, dynamic_computed=, step_sended=WATER=Operative_Level; PIPE_QoS=Operative_Level;, id_entity=135, id_project=38, id_type=32, name_type=Pipe, color=#78C6FA}
      mask prompts: Parameter1 "entity name"; Parameter2 "sampling time"; Parameter3 "project"; resources "input resources and state variables"; Parameter10 "Bring state variables to output"; codeupdate "update code from mask"
      mask help: This is a level-2 MATLAB file S-function which demonstrates CISIA entity
      mask DialogControl Container1 Prompt: All parameters
      mask Display: image('Icons/Pipe.png')
  Pipe_Ward (127) : M-S-Function  FunctionName=cisia_msfun  Parameters=Parameter1, Parameter2, Parameter3, resources, Parameter10, codeupdate, step_received, step_computed, dynamic_computed, step_sended, id_entity, id_project, id_type, name_type, color  mask(S-function:msfcn_unit_delay){Parameter1='Pipe_Ward', Parameter2=1, Parameter3='ORO', resources=*** INPUT RESOURCES *** NUM_INPUTS 1 WATER (1)  *** STATE VARIABLES *** NUM_VARIABLES 3 Operative_Level(NUMERIC)(1)(1) Mechanical_Fault(NUMERIC)(1)(0) Water_Fault(NUMERIC)(1)(0)  *** OUTPUT RESOURCES *** NUM_OUTPUTS 2 WATER (1) PIPE_QoS (1), Parameter10=off, codeupdate=off, step_received=Water_Fault= 1- WATER; Operative_Level=(1-Mechanical_Fault)*(1-0.5*Water_Fault);, step_computed=, dynamic_computed=, step_sended=WATER=Operative_Level; PIPE_QoS=Operative_Level;, id_entity=127, id_project=38, id_type=32, name_type=Pipe, color=#78C6FA}
      mask prompts: Parameter1 "entity name"; Parameter2 "sampling time"; Parameter3 "project"; resources "input resources and state variables"; Parameter10 "Bring state variables to output"; codeupdate "update code from mask"
      mask help: This is a level-2 MATLAB file S-function which demonstrates CISIA entity
      mask DialogControl Container1 Prompt: All parameters
      mask Display: image('Icons/Pipe.png')
  PowerGen_1 (46) : M-S-Function  FunctionName=cisia_msfun  Parameters=Parameter1, Parameter2, Parameter3, resources, Parameter10, codeupdate, step_received, step_computed, dynamic_computed, step_sended, id_entity, id_project, id_type, name_type, color  mask(S-function:msfcn_unit_delay){Parameter1='PowerGen_1', Parameter2=1, Parameter3='ORO', resources=*** INPUT RESOURCES *** NUM_INPUTS 0  *** STATE VARIABLES *** NUM_VARIABLES 2 Operative_Level(NUMERIC)(1)(1) Power_Fault(NUMERIC)(1)(0)  *** OUTPUT RESOURCES *** NUM_OUTPUTS 1 POWER (1), Parameter10=off, codeupdate=off, step_received=Operative_Level=1-Power_Fault;, step_computed=, dynamic_computed=, step_sended=POWER=Operative_Level;, id_entity=46, id_project=38, id_type=8, name_type=PowerSource, color=#84BD8C}
      mask prompts: Parameter1 "entity name"; Parameter2 "sampling time"; Parameter3 "project"; resources "input resources and state variables"; Parameter10 "Bring state variables to output"; codeupdate "update code from mask"
      mask help: This is a level-2 MATLAB file S-function which demonstrates CISIA entity
      mask DialogControl Container1 Prompt: All parameters
      mask Display: image('Icons/PowerSource.png')
  PowerGen_10 (293) : M-S-Function  FunctionName=cisia_msfun  Parameters=Parameter1, Parameter2, Parameter3, resources, Parameter10, codeupdate, step_received, step_computed, dynamic_computed, step_sended, id_entity, id_project, id_type, name_type, color  mask(S-function:msfcn_unit_delay){Parameter1='PowerGen_10', Parameter2=1, Parameter3='ORO', resources=*** INPUT RESOURCES *** NUM_INPUTS 0  *** STATE VARIABLES *** NUM_VARIABLES 2 Operative_Level(NUMERIC)(1)(1) Power_Fault(NUMERIC)(1)(0)  *** OUTPUT RESOURCES *** NUM_OUTPUTS 1 POWER (1), Parameter10=off, codeupdate=off, step_received=Operative_Level=1-Power_Fault;, step_computed=, dynamic_computed=, step_sended=POWER=Operative_Level;, id_entity=293, id_project=38, id_type=8, name_type=PowerSource, color=#84BD8C}
      mask prompts: Parameter1 "entity name"; Parameter2 "sampling time"; Parameter3 "project"; resources "input resources and state variables"; Parameter10 "Bring state variables to output"; codeupdate "update code from mask"
      mask help: This is a level-2 MATLAB file S-function which demonstrates CISIA entity
      mask DialogControl Container1 Prompt: All parameters
      mask Display: image('Icons/PowerSource.png')
  PowerGen_2 (47) : M-S-Function  FunctionName=cisia_msfun  Parameters=Parameter1, Parameter2, Parameter3, resources, Parameter10, codeupdate, step_received, step_computed, dynamic_computed, step_sended, id_entity, id_project, id_type, name_type, color  mask(S-function:msfcn_unit_delay){Parameter1='PowerGen_2', Parameter2=1, Parameter3='ORO', resources=*** INPUT RESOURCES *** NUM_INPUTS 0  *** STATE VARIABLES *** NUM_VARIABLES 2 Operative_Level(NUMERIC)(1)(1) Power_Fault(NUMERIC)(1)(0)  *** OUTPUT RESOURCES *** NUM_OUTPUTS 1 POWER (1), Parameter10=off, codeupdate=off, step_received=Operative_Level=1-Power_Fault;, step_computed=, dynamic_computed=, step_sended=POWER=Operative_Level;, id_entity=47, id_project=38, id_type=8, name_type=PowerSource, color=#84BD8C}
      mask prompts: Parameter1 "entity name"; Parameter2 "sampling time"; Parameter3 "project"; resources "input resources and state variables"; Parameter10 "Bring state variables to output"; codeupdate "update code from mask"
      mask help: This is a level-2 MATLAB file S-function which demonstrates CISIA entity
      mask DialogControl Container1 Prompt: All parameters
      mask Display: image('Icons/PowerSource.png')
  PowerGen_3 (157) : M-S-Function  FunctionName=cisia_msfun  Parameters=Parameter1, Parameter2, Parameter3, resources, Parameter10, codeupdate, step_received, step_computed, dynamic_computed, step_sended, id_entity, id_project, id_type, name_type, color  mask(S-function:msfcn_unit_delay){Parameter1='PowerGen_3', Parameter2=1, Parameter3='ORO', resources=*** INPUT RESOURCES *** NUM_INPUTS 0  *** STATE VARIABLES *** NUM_VARIABLES 2 Operative_Level(NUMERIC)(1)(1) Power_Fault(NUMERIC)(1)(0)  *** OUTPUT RESOURCES *** NUM_OUTPUTS 1 POWER (1), Parameter10=off, codeupdate=off, step_received=Operative_Level=1-Power_Fault;, step_computed=, dynamic_computed=, step_sended=POWER=Operative_Level;, id_entity=157, id_project=38, id_type=8, name_type=PowerSource, color=#84BD8C}
      mask prompts: Parameter1 "entity name"; Parameter2 "sampling time"; Parameter3 "project"; resources "input resources and state variables"; Parameter10 "Bring state variables to output"; codeupdate "update code from mask"
      mask help: This is a level-2 MATLAB file S-function which demonstrates CISIA entity
      mask DialogControl Container1 Prompt: All parameters
      mask Display: image('Icons/PowerSource.png')
  PowerGen_4 (214) : M-S-Function  FunctionName=cisia_msfun  Parameters=Parameter1, Parameter2, Parameter3, resources, Parameter10, codeupdate, step_received, step_computed, dynamic_computed, step_sended, id_entity, id_project, id_type, name_type, color  mask(S-function:msfcn_unit_delay){Parameter1='PowerGen_4', Parameter2=1, Parameter3='ORO', resources=*** INPUT RESOURCES *** NUM_INPUTS 0  *** STATE VARIABLES *** NUM_VARIABLES 2 Operative_Level(NUMERIC)(1)(1) Power_Fault(NUMERIC)(1)(0)  *** OUTPUT RESOURCES *** NUM_OUTPUTS 1 POWER (1), Parameter10=off, codeupdate=off, step_received=Operative_Level=1-Power_Fault;, step_computed=, dynamic_computed=, step_sended=POWER=Operative_Level;, id_entity=214, id_project=38, id_type=8, name_type=PowerSource, color=#84BD8C}
      mask prompts: Parameter1 "entity name"; Parameter2 "sampling time"; Parameter3 "project"; resources "input resources and state variables"; Parameter10 "Bring state variables to output"; codeupdate "update code from mask"
      mask help: This is a level-2 MATLAB file S-function which demonstrates CISIA entity
      mask DialogControl Container1 Prompt: All parameters
      mask Display: image('Icons/PowerSource.png')
  PowerGen_5 (236) : M-S-Function  FunctionName=cisia_msfun  Parameters=Parameter1, Parameter2, Parameter3, resources, Parameter10, codeupdate, step_received, step_computed, dynamic_computed, step_sended, id_entity, id_project, id_type, name_type, color  mask(S-function:msfcn_unit_delay){Parameter1='PowerGen_5', Parameter2=1, Parameter3='ORO', resources=*** INPUT RESOURCES *** NUM_INPUTS 0  *** STATE VARIABLES *** NUM_VARIABLES 2 Operative_Level(NUMERIC)(1)(1) Power_Fault(NUMERIC)(1)(0)  *** OUTPUT RESOURCES *** NUM_OUTPUTS 1 POWER (1), Parameter10=off, codeupdate=off, step_received=Operative_Level=1-Power_Fault;, step_computed=, dynamic_computed=, step_sended=POWER=Operative_Level;, id_entity=236, id_project=38, id_type=8, name_type=PowerSource, color=#84BD8C}
      mask prompts: Parameter1 "entity name"; Parameter2 "sampling time"; Parameter3 "project"; resources "input resources and state variables"; Parameter10 "Bring state variables to output"; codeupdate "update code from mask"
      mask help: This is a level-2 MATLAB file S-function which demonstrates CISIA entity
      mask DialogControl Container1 Prompt: All parameters
      mask Display: image('Icons/PowerSource.png')
  PowerGen_6 (245) : M-S-Function  FunctionName=cisia_msfun  Parameters=Parameter1, Parameter2, Parameter3, resources, Parameter10, codeupdate, step_received, step_computed, dynamic_computed, step_sended, id_entity, id_project, id_type, name_type, color  mask(S-function:msfcn_unit_delay){Parameter1='PowerGen_6', Parameter2=1, Parameter3='ORO', resources=*** INPUT RESOURCES *** NUM_INPUTS 0  *** STATE VARIABLES *** NUM_VARIABLES 2 Operative_Level(NUMERIC)(1)(1) Power_Fault(NUMERIC)(1)(0)  *** OUTPUT RESOURCES *** NUM_OUTPUTS 1 POWER (1), Parameter10=off, codeupdate=off, step_received=Operative_Level=1-Power_Fault;, step_computed=, dynamic_computed=, step_sended=POWER=Operative_Level;, id_entity=245, id_project=38, id_type=8, name_type=PowerSource, color=#84BD8C}
      mask prompts: Parameter1 "entity name"; Parameter2 "sampling time"; Parameter3 "project"; resources "input resources and state variables"; Parameter10 "Bring state variables to output"; codeupdate "update code from mask"
      mask help: This is a level-2 MATLAB file S-function which demonstrates CISIA entity
      mask DialogControl Container1 Prompt: All parameters
      mask Display: image('Icons/PowerSource.png')
  PowerGen_7 (260) : M-S-Function  FunctionName=cisia_msfun  Parameters=Parameter1, Parameter2, Parameter3, resources, Parameter10, codeupdate, step_received, step_computed, dynamic_computed, step_sended, id_entity, id_project, id_type, name_type, color  mask(S-function:msfcn_unit_delay){Parameter1='PowerGen_7', Parameter2=1, Parameter3='ORO', resources=*** INPUT RESOURCES *** NUM_INPUTS 0  *** STATE VARIABLES *** NUM_VARIABLES 2 Operative_Level(NUMERIC)(1)(1) Power_Fault(NUMERIC)(1)(0)  *** OUTPUT RESOURCES *** NUM_OUTPUTS 1 POWER (1), Parameter10=off, codeupdate=off, step_received=Operative_Level=1-Power_Fault;, step_computed=, dynamic_computed=, step_sended=POWER=Operative_Level;, id_entity=260, id_project=38, id_type=8, name_type=PowerSource, color=#84BD8C}
      mask prompts: Parameter1 "entity name"; Parameter2 "sampling time"; Parameter3 "project"; resources "input resources and state variables"; Parameter10 "Bring state variables to output"; codeupdate "update code from mask"
      mask help: This is a level-2 MATLAB file S-function which demonstrates CISIA entity
      mask DialogControl Container1 Prompt: All parameters
      mask Display: image('Icons/PowerSource.png')
  PowerGen_8 (281) : M-S-Function  FunctionName=cisia_msfun  Parameters=Parameter1, Parameter2, Parameter3, resources, Parameter10, codeupdate, step_received, step_computed, dynamic_computed, step_sended, id_entity, id_project, id_type, name_type, color  mask(S-function:msfcn_unit_delay){Parameter1='PowerGen_8', Parameter2=1, Parameter3='ORO', resources=*** INPUT RESOURCES *** NUM_INPUTS 0  *** STATE VARIABLES *** NUM_VARIABLES 2 Operative_Level(NUMERIC)(1)(1) Power_Fault(NUMERIC)(1)(0)  *** OUTPUT RESOURCES *** NUM_OUTPUTS 1 POWER (1), Parameter10=off, codeupdate=off, step_received=Operative_Level=1-Power_Fault;, step_computed=, dynamic_computed=, step_sended=POWER=Operative_Level;, id_entity=281, id_project=38, id_type=8, name_type=PowerSource, color=#84BD8C}
      mask prompts: Parameter1 "entity name"; Parameter2 "sampling time"; Parameter3 "project"; resources "input resources and state variables"; Parameter10 "Bring state variables to output"; codeupdate "update code from mask"
      mask help: This is a level-2 MATLAB file S-function which demonstrates CISIA entity
      mask DialogControl Container1 Prompt: All parameters
      mask Display: image('Icons/PowerSource.png')
  PowerGen_9 (294) : M-S-Function  FunctionName=cisia_msfun  Parameters=Parameter1, Parameter2, Parameter3, resources, Parameter10, codeupdate, step_received, step_computed, dynamic_computed, step_sended, id_entity, id_project, id_type, name_type, color  mask(S-function:msfcn_unit_delay){Parameter1='PowerGen_9', Parameter2=1, Parameter3='ORO', resources=*** INPUT RESOURCES *** NUM_INPUTS 0  *** STATE VARIABLES *** NUM_VARIABLES 2 Operative_Level(NUMERIC)(1)(1) Power_Fault(NUMERIC)(1)(0)  *** OUTPUT RESOURCES *** NUM_OUTPUTS 1 POWER (1), Parameter10=off, codeupdate=off, step_received=Operative_Level=1-Power_Fault;, step_computed=, dynamic_computed=, step_sended=POWER=Operative_Level;, id_entity=294, id_project=38, id_type=8, name_type=PowerSource, color=#84BD8C}
      mask prompts: Parameter1 "entity name"; Parameter2 "sampling time"; Parameter3 "project"; resources "input resources and state variables"; Parameter10 "Bring state variables to output"; codeupdate "update code from mask"
      mask help: This is a level-2 MATLAB file S-function which demonstrates CISIA entity
      mask DialogControl Container1 Prompt: All parameters
      mask Display: image('Icons/PowerSource.png')
  RESISTO_1 (196) : M-S-Function  FunctionName=cisia_msfun  Parameters=Parameter1, Parameter2, Parameter3, resources, Parameter10, codeupdate, step_received, step_computed, dynamic_computed, step_sended, id_entity, id_project, id_type, name_type, color  mask(S-function:msfcn_unit_delay){Parameter1='RESISTO_1', Parameter2=1, Parameter3='ORO', resources=*** INPUT RESOURCES *** NUM_INPUTS 4 TLC_CONN (20) TLC_SERVICE (20) CYBER_FAULT (10) POWER (1)  *** STATE VARIABLES *** NUM_VARIABLES 18 Operative_Level(NUMERIC)(1)(1) Connection(NUMERIC_ARRAY)(20)(0  0  0  0  0  0  0  0  0  0  0  0  0  0  0  0  0  0  0  0) Dos_attack(NUMERIC)(1)(0) MITM_attack(NUMERIC)(1)(0) Virus_Attack(NUMERIC)(1)(0) Port_Scan_Attack(NUMERIC)(1)(0) Cyber_Fault(NUMERIC_ARRAY)(10)(0  0  0  0  0  0  0  0  0  0) BGP_hijacking(NUMERIC)(1)(0) Mechanical_Fault(NUMERIC)(1)(0) Conn_Fault(NUMERIC)(1)(0) Consumed_Services(NUMERIC_ARRAY)(20)(0  0  0  0  0  0  0  0  0  0  0  0  0  0  0  0  0  0  0  0) Service_Fault(NUMERIC)(1)(0) Redundancy_Fault(NUMERIC)(1)(0) BotNet_Attack(NUMERIC)(1)(0) Data_Corruption(NUMERIC)(1)(0) SW_Change(NUMERIC)(1)(0) Config_Change(NUMERIC)(1)(0) Port_Saturation(NUMERIC)(1)(0)  *** OUTPUT RESOURCES *** NUM_OUTPUTS 1 WORKSTATION_QoS (1), Parameter10=off, codeupdate=off, step_received=Connection=max(Connection_init,TLC_CONN);  Cyber_Fault=max(CYBER_FAULT, transpose([Dos_attack   MITM_attack Virus_Attack Port_Scan_Attack  BGP_hijacking BotNet_Attack Data_Corruption SW_Change Config_Change Port_Saturation]));  % Vale 1 in presenza di fault Conn_Fault=max([Dos_attack  Mechanical_Fault  1-POWER] );    Operative_Level=(1-Conn_Fault)*max(max(TLC_CONN),0.5);, step_computed=, dynamic_computed=, step_sended=WORKSTATION_QoS=Operative_Level;, id_entity=196, id_project=38, id_type=43, name_type=Workstation, color=#FFFFFF}
      mask prompts: Parameter1 "entity name"; Parameter2 "sampling time"; Parameter3 "project"; resources "input resources and state variables"; Parameter10 "Bring state variables to output"; codeupdate "update code from mask"
      mask help: This is a level-2 MATLAB file S-function which demonstrates CISIA entity
      mask DialogControl Container1 Prompt: All parameters
      mask Display: image('Icons/RESISTO_1.png')
  ROBOT_QoS : MinMax  Inputs=2
  ROUTE_TIM_1 (20) : M-S-Function  FunctionName=cisia_msfun  Parameters=Parameter1, Parameter2, Parameter3, Parameter4, Parameter5, Parameter6, Parameter7  mask(S-function:msfcn_unit_delay){Parameter1='ROUTE_TIM_1', Parameter2=1, Parameter3='ORO', Parameter4=9, Parameter5=0, Parameter6=20, Parameter7=off}
      mask prompts: Parameter1 "entity name"; Parameter2 "sampling time"; Parameter3 "project"; Parameter4 "number of output links"; Parameter5 "default value for outputs"; Parameter6 "link dimension (unused))"; Parameter7 "select resource elements and output port from input"
      mask help: This is a level-2 MATLAB file S-function which demonstrates CISIA entity
      mask Display: disp('ROUTE')
  ROUTE_TIM_2 (21) : M-S-Function  FunctionName=cisia_msfun  Parameters=Parameter1, Parameter2, Parameter3, Parameter4, Parameter5, Parameter6, Parameter7  mask(S-function:msfcn_unit_delay){Parameter1='ROUTE_TIM_2', Parameter2=1, Parameter3='ORO', Parameter4=9, Parameter5=0, Parameter6=20, Parameter7=off}
      mask prompts: Parameter1 "entity name"; Parameter2 "sampling time"; Parameter3 "project"; Parameter4 "number of output links"; Parameter5 "default value for outputs"; Parameter6 "link dimension (unused))"; Parameter7 "select resource elements and output port from input"
      mask help: This is a level-2 MATLAB file S-function which demonstrates CISIA entity
      mask Display: disp('ROUTE')
  ROUTE_TIM_3 (22) : M-S-Function  FunctionName=cisia_msfun  Parameters=Parameter1, Parameter2, Parameter3, Parameter4, Parameter5, Parameter6, Parameter7  mask(S-function:msfcn_unit_delay){Parameter1='ROUTE_TIM_3', Parameter2=1, Parameter3='ORO', Parameter4=2, Parameter5=0, Parameter6=20, Parameter7=off}
      mask prompts: Parameter1 "entity name"; Parameter2 "sampling time"; Parameter3 "project"; Parameter4 "number of output links"; Parameter5 "default value for outputs"; Parameter6 "link dimension (unused))"; Parameter7 "select resource elements and output port from input"
      mask help: This is a level-2 MATLAB file S-function which demonstrates CISIA entity
      mask Display: disp('ROUTE')
  ROUTE_TIM_4 (23) : M-S-Function  FunctionName=cisia_msfun  Parameters=Parameter1, Parameter2, Parameter3, Parameter4, Parameter5, Parameter6, Parameter7  mask(S-function:msfcn_unit_delay){Parameter1='ROUTE_TIM_4', Parameter2=1, Parameter3='ORO', Parameter4=2, Parameter5=0, Parameter6=20, Parameter7=off}
      mask prompts: Parameter1 "entity name"; Parameter2 "sampling time"; Parameter3 "project"; Parameter4 "number of output links"; Parameter5 "default value for outputs"; Parameter6 "link dimension (unused))"; Parameter7 "select resource elements and output port from input"
      mask help: This is a level-2 MATLAB file S-function which demonstrates CISIA entity
      mask Display: disp('ROUTE')
  R_Wire_1 (98) : M-S-Function  FunctionName=cisia_msfun  Parameters=Parameter1, Parameter2, Parameter3, resources, Parameter10, codeupdate, step_received, step_computed, dynamic_computed, step_sended, id_entity, id_project, id_type, name_type, color  mask(S-function:msfcn_unit_delay){Parameter1='R_Wire_1', Parameter2=1, Parameter3='ORO', resources=*** INPUT RESOURCES *** NUM_INPUTS 4 TLC_CONN (20) TLC_SERVICE (20) CYBER_FAULT (10) MECH_FAULT (1)  *** STATE VARIABLES *** NUM_VARIABLES 8 Operative_Level(NUMERIC)(1)(1) TLC_services(NUMERIC_ARRAY)(20)(0  0  0  0  0  0  0  0  0  0  0  0  0  0  0  0  0  0  0  0) Connection(NUMERIC_ARRAY)(20)(0  0  0  0  0  0  0  0  0  0  0  0  0  0  0  0  0  0  0  0) Dos_attack(NUMERIC)(1)(0) Cyber_Fault(NUMERIC_ARRAY)(10)(0  0  0  0  0  0  0  0  0  0) Mechanical_Fault(NUMERIC)(1)(0) Conn_Fault(NUMERIC)(1)(0) TLC_revoke(NUMERIC_ARRAY)(20)(0  0  0  0  0  0  0  0  0  0  0  0  0  0  0  0  0  0  0  0)  *** OUTPUT RESOURCES *** NUM_OUTPUTS 4 TLC_CONN (20) TLC_SERVICE (20) CYBER_FAULT (10) MECH_FAULT (1), Parameter10=off, codeupdate=off, step_received=Connection=max(Connection_init,TLC_CONN); TLC_services=max(TLC_services_init,TLC_SERVICE); TLC_services=mod(TLC_services,10); TLC_revoke=floor(TLC_SERVICE/10);  Cyber_Fault=CYBER_FAULT;  Mechanical_Fault=max([Mechanical_Fault MECH_FAULT Mechanical_Fault_init]);  %TLC_services=TLC_services.*(1-TLC_revoke);  Operative_Level=1-Mechanical_Fault;, step_computed=, dynamic_computed=, step_sended=TLC_CONN=Connection*Operative_Level; TLC_SERVICE=TLC_services*Operative_Level+10*TLC_revoke; CYBER_FAULT=Cyber_Fault*Operative_Level; MECH_FAULT=Mechanical_Fault;, id_entity=98, id_project=38, id_type=21, name_type=Redundant_Wire, color=#038F03}
      mask prompts: Parameter1 "entity name"; Parameter2 "sampling time"; Parameter3 "project"; resources "input resources and state variables"; Parameter10 "Bring state variables to output"; codeupdate "update code from mask"
      mask help: This is a level-2 MATLAB file S-function which demonstrates CISIA entity
      mask DialogControl Container1 Prompt: All parameters
      mask Display: disp('Redundant_Wire')
  R_Wire_1b (99) : M-S-Function  FunctionName=cisia_msfun  Parameters=Parameter1, Parameter2, Parameter3, resources, Parameter10, codeupdate, step_received, step_computed, dynamic_computed, step_sended, id_entity, id_project, id_type, name_type, color  mask(S-function:msfcn_unit_delay){Parameter1='R_Wire_1b', Parameter2=1, Parameter3='ORO', resources=*** INPUT RESOURCES *** NUM_INPUTS 4 TLC_CONN (20) TLC_SERVICE (20) CYBER_FAULT (10) MECH_FAULT (1)  *** STATE VARIABLES *** NUM_VARIABLES 8 Operative_Level(NUMERIC)(1)(1) TLC_services(NUMERIC_ARRAY)(20)(0  0  0  0  0  0  0  0  0  0  0  0  0  0  0  0  0  0  0  0) Connection(NUMERIC_ARRAY)(20)(0  0  0  0  0  0  0  0  0  0  0  0  0  0  0  0  0  0  0  0) Dos_attack(NUMERIC)(1)(0) Cyber_Fault(NUMERIC_ARRAY)(10)(0  0  0  0  0  0  0  0  0  0) Mechanical_Fault(NUMERIC)(1)(0) Conn_Fault(NUMERIC)(1)(0) TLC_revoke(NUMERIC_ARRAY)(20)(0  0  0  0  0  0  0  0  0  0  0  0  0  0  0  0  0  0  0  0)  *** OUTPUT RESOURCES *** NUM_OUTPUTS 4 TLC_CONN (20) TLC_SERVICE (20) CYBER_FAULT (10) MECH_FAULT (1), Parameter10=off, codeupdate=off, step_received=Connection=max(Connection_init,TLC_CONN); TLC_services=max(TLC_services_init,TLC_SERVICE); TLC_services=mod(TLC_services,10); TLC_revoke=floor(TLC_SERVICE/10);  Cyber_Fault=CYBER_FAULT;  Mechanical_Fault=max([Mechanical_Fault MECH_FAULT Mechanical_Fault_init]);  %TLC_services=TLC_services.*(1-TLC_revoke);  Operative_Level=1-Mechanical_Fault;, step_computed=, dynamic_computed=, step_sended=TLC_CONN=Connection*Operative_Level; TLC_SERVICE=TLC_services*Operative_Level+10*TLC_revoke; CYBER_FAULT=Cyber_Fault*Operative_Level; MECH_FAULT=Mechanical_Fault;, id_entity=99, id_project=38, id_type=21, name_type=Redundant_Wire, color=#038F03}
      mask prompts: Parameter1 "entity name"; Parameter2 "sampling time"; Parameter3 "project"; resources "input resources and state variables"; Parameter10 "Bring state variables to output"; codeupdate "update code from mask"
      mask help: This is a level-2 MATLAB file S-function which demonstrates CISIA entity
      mask DialogControl Container1 Prompt: All parameters
      mask Display: disp('Redundant_Wire')
  Robot_1 (203) : M-S-Function  FunctionName=cisia_msfun  Parameters=Parameter1, Parameter2, Parameter3, resources, Parameter10, codeupdate, step_received, step_computed, dynamic_computed, step_sended, id_entity, id_project, id_type, name_type, color  mask(S-function:msfcn_unit_delay){Parameter1='Robot_1', Parameter2=1, Parameter3='ORO', resources=*** INPUT RESOURCES *** NUM_INPUTS 3 TLC_SERVICE (20) POWER (1) R_CONN (20)  *** STATE VARIABLES *** NUM_VARIABLES 12 Operative_Level(NUMERIC)(1)(1) TLC_services(NUMERIC_ARRAY)(20)(0  0  0  0  0  0  0  0  0  0  0  0  0  0  0  0  0  0  0  0) Connection(NUMERIC_ARRAY)(20)(0  0  0  0  0  0  0  0  0  0  0  0  0  0  0  0  0  0  0  0) Mechanical_Fault(NUMERIC)(1)(0) Consumed_Services(NUMERIC_ARRAY)(20)(0  0  0  0  1  0  0  0  1  0  0  0  0  0  0  0  0  0  0  0) Service_Fault(NUMERIC)(1)(0) Redundancy_Fault(NUMERIC)(1)(0) Physical_Fault(NUMERIC)(1)(0) TLC_revoke(NUMERIC_ARRAY)(20)(0  0  0  0  0  0  0  0  0  0  0  0  0  0  0  0  0  0  0  0) Alternative_Services(NUMERIC_ARRAY)(20)(0  0  0  0  0  1  0  0  0  1  0  0  0  0  0  0  0  0  0  0) Alt_Serv_Fault(NUMERIC)(1)(0) Alt_Rout_Fault(NUMERIC)(1)(0)  *** OUTPUT RESOURCES *** NUM_OUTPUTS 3 ROBOT_QoS (1) ALT_ROUTING (1) ALT_SERVICES (1), Parameter10=off, codeupdate=off, step_received=Connection=max(Connection_init,R_CONN); TLC_services=max(TLC_services_init,TLC_SERVICE); TLC_services=mod(TLC_services,10); TLC_revoke=floor(TLC_SERVICE/10);  Physical_Fault=max([Mechanical_Fault  1-POWER] );  Service_Fault=max(abs(Consumed_Services.*TLC_services-Consumed_Services)); Redundancy_Fault=max(abs(Consumed_Services.*R_CONN-Consumed_Services));   Alt_Serv_Fault=max(abs(Alternative_Services.*R_CONN-Alternative_Services));  Alt_Rout_Fault=max(abs(Consumed_Services.*R_CONN-Consumed_Services));   Operative_Level=(1-Physical_Fault)*max(max(R_CONN),0.5)*(1-0.6*Service_Fault);, step_computed=, dynamic_computed=, step_sended=ROBOT_QoS=Operative_Level;   ALT_SERVICES=1-Alt_Serv_Fault; ALT_ROUTING=1-Alt_Rout_Fault;, id_entity=203, id_project=38, id_type=44, name_type=Robot, color=#FFFFFF}
      mask prompts: Parameter1 "entity name"; Parameter2 "sampling time"; Parameter3 "project"; resources "input resources and state variables"; Parameter10 "Bring state variables to output"; codeupdate "update code from mask"
      mask help: This is a level-2 MATLAB file S-function which demonstrates CISIA entity
      mask DialogControl Container1 Prompt: All parameters
      mask Display: image('Icons/Robot.png')
  Robot_2 (205) : M-S-Function  FunctionName=cisia_msfun  Parameters=Parameter1, Parameter2, Parameter3, resources, Parameter10, codeupdate, step_received, step_computed, dynamic_computed, step_sended, id_entity, id_project, id_type, name_type, color  mask(S-function:msfcn_unit_delay){Parameter1='Robot_2', Parameter2=1, Parameter3='ORO', resources=*** INPUT RESOURCES *** NUM_INPUTS 3 TLC_SERVICE (20) POWER (1) R_CONN (20)  *** STATE VARIABLES *** NUM_VARIABLES 12 Operative_Level(NUMERIC)(1)(1) TLC_services(NUMERIC_ARRAY)(20)(0  0  0  0  0  0  0  0  0  0  0  0  0  0  0  0  0  0  0  0) Connection(NUMERIC_ARRAY)(20)(0  0  0  0  0  0  0  0  0  0  0  0  0  0  0  0  0  0  0  0) Mechanical_Fault(NUMERIC)(1)(0) Consumed_Services(NUMERIC_ARRAY)(20)(0  0  0  0  1  0  0  0  1  0  0  0  0  0  0  0  0  0  0  0) Service_Fault(NUMERIC)(1)(0) Redundancy_Fault(NUMERIC)(1)(0) Physical_Fault(NUMERIC)(1)(0) TLC_revoke(NUMERIC_ARRAY)(20)(0  0  0  0  0  0  0  0  0  0  0  0  0  0  0  0  0  0  0  0) Alternative_Services(NUMERIC_ARRAY)(20)(0  0  0  0  0  1  0  0  0  1  0  0  0  0  0  0  0  0  0  0) Alt_Serv_Fault(NUMERIC)(1)(0) Alt_Rout_Fault(NUMERIC)(1)(0)  *** OUTPUT RESOURCES *** NUM_OUTPUTS 3 ROBOT_QoS (1) ALT_ROUTING (1) ALT_SERVICES (1), Parameter10=off, codeupdate=off, step_received=Connection=max(Connection_init,R_CONN); TLC_services=max(TLC_services_init,TLC_SERVICE); TLC_services=mod(TLC_services,10); TLC_revoke=floor(TLC_SERVICE/10);  Physical_Fault=max([Mechanical_Fault  1-POWER] );  Service_Fault=max(abs(Consumed_Services.*TLC_services-Consumed_Services)); Redundancy_Fault=max(abs(Consumed_Services.*R_CONN-Consumed_Services));   Alt_Serv_Fault=max(abs(Alternative_Services.*R_CONN-Alternative_Services));  Alt_Rout_Fault=max(abs(Consumed_Services.*R_CONN-Consumed_Services));   Operative_Level=(1-Physical_Fault)*max(max(R_CONN),0.5)*(1-0.6*Service_Fault);, step_computed=, dynamic_computed=, step_sended=ROBOT_QoS=Operative_Level;   ALT_SERVICES=1-Alt_Serv_Fault; ALT_ROUTING=1-Alt_Rout_Fault;, id_entity=205, id_project=38, id_type=44, name_type=Robot, color=#FFFFFF}
      mask prompts: Parameter1 "entity name"; Parameter2 "sampling time"; Parameter3 "project"; resources "input resources and state variables"; Parameter10 "Bring state variables to output"; codeupdate "update code from mask"
      mask help: This is a level-2 MATLAB file S-function which demonstrates CISIA entity
      mask DialogControl Container1 Prompt: All parameters
      mask Display: image('Icons/Robot.png')
  Room_1 (51) : M-S-Function  FunctionName=cisia_msfun  Parameters=Parameter1, Parameter2, Parameter3, resources, Parameter10, codeupdate, step_received, step_computed, dynamic_computed, step_sended, id_entity, id_project, id_type, name_type, color  mask(S-function:msfcn_unit_delay){Parameter1='Room_1', Parameter2=1, Parameter3='ORO', resources=*** INPUT RESOURCES *** NUM_INPUTS 1 POWER (1)  *** STATE VARIABLES *** NUM_VARIABLES 8 Operative_Level(NUMERIC)(1)(1) Power_Fault(NUMERIC)(1)(0) Cooling_Fault(NUMERIC)(1)(0) Flooding_Fault(NUMERIC)(1)(0) Fire_Fault(NUMERIC)(1)(0) Unauthorized_Access(NUMERIC)(1)(0) Earthquake_Fault(NUMERIC)(1)(0) Physical_Fault(NUMERIC)(1)(0)  *** OUTPUT RESOURCES *** NUM_OUTPUTS 1 ROOM_QoS (1), Parameter10=off, codeupdate=off, step_received=Physical_Fault=max([Power_Fault Flooding_Fault Fire_Fault Cooling_Fault 1-POWER]);   %Operative_Level=min([1-Power_Fault 1-Flooding_Fault  1-Fire_Fault  1-Cooling_Fault  POWER]); %Operative_Level=Operative_Level*max((1-Unauthorized_Access),0.5);  Operative_Level=(1-Physical_Fault)*(1-0.5*Unauthorized_Access);, step_computed=, dynamic_computed=, step_sended=ROOM_QoS=Operative_Level;, id_entity=51, id_project=38, id_type=9, name_type=Room, color=#EDB120}
      mask prompts: Parameter1 "entity name"; Parameter2 "sampling time"; Parameter3 "project"; resources "input resources and state variables"; Parameter10 "Bring state variables to output"; codeupdate "update code from mask"
      mask help: This is a level-2 MATLAB file S-function which demonstrates CISIA entity
      mask DialogControl Container1 Prompt: All parameters
      mask Display: image('Icons/Room.png')
  Room_10 (257) : M-S-Function  FunctionName=cisia_msfun  Parameters=Parameter1, Parameter2, Parameter3, resources, Parameter10, codeupdate, step_received, step_computed, dynamic_computed, step_sended, id_entity, id_project, id_type, name_type, color  mask(S-function:msfcn_unit_delay){Parameter1='Room_10', Parameter2=1, Parameter3='ORO', resources=*** INPUT RESOURCES *** NUM_INPUTS 1 POWER (1)  *** STATE VARIABLES *** NUM_VARIABLES 8 Operative_Level(NUMERIC)(1)(1) Power_Fault(NUMERIC)(1)(0) Cooling_Fault(NUMERIC)(1)(0) Flooding_Fault(NUMERIC)(1)(0) Fire_Fault(NUMERIC)(1)(0) Unauthorized_Access(NUMERIC)(1)(0) Earthquake_Fault(NUMERIC)(1)(0) Physical_Fault(NUMERIC)(1)(0)  *** OUTPUT RESOURCES *** NUM_OUTPUTS 1 ROOM_QoS (1), Parameter10=off, codeupdate=off, step_received=Physical_Fault=max([Power_Fault Flooding_Fault Fire_Fault Cooling_Fault 1-POWER]);   %Operative_Level=min([1-Power_Fault 1-Flooding_Fault  1-Fire_Fault  1-Cooling_Fault  POWER]); %Operative_Level=Operative_Level*max((1-Unauthorized_Access),0.5);  Operative_Level=(1-Physical_Fault)*(1-0.5*Unauthorized_Access);, step_computed=, dynamic_computed=, step_sended=ROOM_QoS=Operative_Level;, id_entity=257, id_project=38, id_type=9, name_type=Room, color=#EDB120}
      mask prompts: Parameter1 "entity name"; Parameter2 "sampling time"; Parameter3 "project"; resources "input resources and state variables"; Parameter10 "Bring state variables to output"; codeupdate "update code from mask"
      mask help: This is a level-2 MATLAB file S-function which demonstrates CISIA entity
      mask DialogControl Container1 Prompt: All parameters
      mask Display: image('Icons/Room.png')
  Room_11 (258) : M-S-Function  FunctionName=cisia_msfun  Parameters=Parameter1, Parameter2, Parameter3, resources, Parameter10, codeupdate, step_received, step_computed, dynamic_computed, step_sended, id_entity, id_project, id_type, name_type, color  mask(S-function:msfcn_unit_delay){Parameter1='Room_11', Parameter2=1, Parameter3='ORO', resources=*** INPUT RESOURCES *** NUM_INPUTS 1 POWER (1)  *** STATE VARIABLES *** NUM_VARIABLES 8 Operative_Level(NUMERIC)(1)(1) Power_Fault(NUMERIC)(1)(0) Cooling_Fault(NUMERIC)(1)(0) Flooding_Fault(NUMERIC)(1)(0) Fire_Fault(NUMERIC)(1)(0) Unauthorized_Access(NUMERIC)(1)(0) Earthquake_Fault(NUMERIC)(1)(0) Physical_Fault(NUMERIC)(1)(0)  *** OUTPUT RESOURCES *** NUM_OUTPUTS 1 ROOM_QoS (1), Parameter10=off, codeupdate=off, step_received=Physical_Fault=max([Power_Fault Flooding_Fault Fire_Fault Cooling_Fault 1-POWER]);   %Operative_Level=min([1-Power_Fault 1-Flooding_Fault  1-Fire_Fault  1-Cooling_Fault  POWER]); %Operative_Level=Operative_Level*max((1-Unauthorized_Access),0.5);  Operative_Level=(1-Physical_Fault)*(1-0.5*Unauthorized_Access);, step_computed=, dynamic_computed=, step_sended=ROOM_QoS=Operative_Level;, id_entity=258, id_project=38, id_type=9, name_type=Room, color=#EDB120}
      mask prompts: Parameter1 "entity name"; Parameter2 "sampling time"; Parameter3 "project"; resources "input resources and state variables"; Parameter10 "Bring state variables to output"; codeupdate "update code from mask"
      mask help: This is a level-2 MATLAB file S-function which demonstrates CISIA entity
      mask DialogControl Container1 Prompt: All parameters
      mask Display: image('Icons/Room.png')
  Room_12 (259) : M-S-Function  FunctionName=cisia_msfun  Parameters=Parameter1, Parameter2, Parameter3, resources, Parameter10, codeupdate, step_received, step_computed, dynamic_computed, step_sended, id_entity, id_project, id_type, name_type, color  mask(S-function:msfcn_unit_delay){Parameter1='Room_12', Parameter2=1, Parameter3='ORO', resources=*** INPUT RESOURCES *** NUM_INPUTS 1 POWER (1)  *** STATE VARIABLES *** NUM_VARIABLES 8 Operative_Level(NUMERIC)(1)(1) Power_Fault(NUMERIC)(1)(0) Cooling_Fault(NUMERIC)(1)(0) Flooding_Fault(NUMERIC)(1)(0) Fire_Fault(NUMERIC)(1)(0) Unauthorized_Access(NUMERIC)(1)(0) Earthquake_Fault(NUMERIC)(1)(0) Physical_Fault(NUMERIC)(1)(0)  *** OUTPUT RESOURCES *** NUM_OUTPUTS 1 ROOM_QoS (1), Parameter10=off, codeupdate=off, step_received=Physical_Fault=max([Power_Fault Flooding_Fault Fire_Fault Cooling_Fault 1-POWER]);   %Operative_Level=min([1-Power_Fault 1-Flooding_Fault  1-Fire_Fault  1-Cooling_Fault  POWER]); %Operative_Level=Operative_Level*max((1-Unauthorized_Access),0.5);  Operative_Level=(1-Physical_Fault)*(1-0.5*Unauthorized_Access);, step_computed=, dynamic_computed=, step_sended=ROOM_QoS=Operative_Level;, id_entity=259, id_project=38, id_type=9, name_type=Room, color=#EDB120}
      mask prompts: Parameter1 "entity name"; Parameter2 "sampling time"; Parameter3 "project"; resources "input resources and state variables"; Parameter10 "Bring state variables to output"; codeupdate "update code from mask"
      mask help: This is a level-2 MATLAB file S-function which demonstrates CISIA entity
      mask DialogControl Container1 Prompt: All parameters
      mask Display: image('Icons/Room.png')
  Room_13 (262) : M-S-Function  FunctionName=cisia_msfun  Parameters=Parameter1, Parameter2, Parameter3, resources, Parameter10, codeupdate, step_received, step_computed, dynamic_computed, step_sended, id_entity, id_project, id_type, name_type, color  mask(S-function:msfcn_unit_delay){Parameter1='Room_13', Parameter2=1, Parameter3='ORO', resources=*** INPUT RESOURCES *** NUM_INPUTS 1 POWER (1)  *** STATE VARIABLES *** NUM_VARIABLES 8 Operative_Level(NUMERIC)(1)(1) Power_Fault(NUMERIC)(1)(0) Cooling_Fault(NUMERIC)(1)(0) Flooding_Fault(NUMERIC)(1)(0) Fire_Fault(NUMERIC)(1)(0) Unauthorized_Access(NUMERIC)(1)(0) Earthquake_Fault(NUMERIC)(1)(0) Physical_Fault(NUMERIC)(1)(0)  *** OUTPUT RESOURCES *** NUM_OUTPUTS 1 ROOM_QoS (1), Parameter10=off, codeupdate=off, step_received=Physical_Fault=max([Power_Fault Flooding_Fault Fire_Fault Cooling_Fault 1-POWER]);   %Operative_Level=min([1-Power_Fault 1-Flooding_Fault  1-Fire_Fault  1-Cooling_Fault  POWER]); %Operative_Level=Operative_Level*max((1-Unauthorized_Access),0.5);  Operative_Level=(1-Physical_Fault)*(1-0.5*Unauthorized_Access);, step_computed=, dynamic_computed=, step_sended=ROOM_QoS=Operative_Level;, id_entity=262, id_project=38, id_type=9, name_type=Room, color=#EDB120}
      mask prompts: Parameter1 "entity name"; Parameter2 "sampling time"; Parameter3 "project"; resources "input resources and state variables"; Parameter10 "Bring state variables to output"; codeupdate "update code from mask"
      mask help: This is a level-2 MATLAB file S-function which demonstrates CISIA entity
      mask DialogControl Container1 Prompt: All parameters
      mask Display: image('Icons/Room.png')
  Room_14 (284) : M-S-Function  FunctionName=cisia_msfun  Parameters=Parameter1, Parameter2, Parameter3, resources, Parameter10, codeupdate, step_received, step_computed, dynamic_computed, step_sended, id_entity, id_project, id_type, name_type, color  mask(S-function:msfcn_unit_delay){Parameter1='Room_14', Parameter2=1, Parameter3='ORO', resources=*** INPUT RESOURCES *** NUM_INPUTS 1 POWER (1)  *** STATE VARIABLES *** NUM_VARIABLES 8 Operative_Level(NUMERIC)(1)(1) Power_Fault(NUMERIC)(1)(0) Cooling_Fault(NUMERIC)(1)(0) Flooding_Fault(NUMERIC)(1)(0) Fire_Fault(NUMERIC)(1)(0) Unauthorized_Access(NUMERIC)(1)(0) Earthquake_Fault(NUMERIC)(1)(0) Physical_Fault(NUMERIC)(1)(0)  *** OUTPUT RESOURCES *** NUM_OUTPUTS 1 ROOM_QoS (1), Parameter10=off, codeupdate=off, step_received=Physical_Fault=max([Power_Fault Flooding_Fault Fire_Fault Cooling_Fault 1-POWER]);   %Operative_Level=min([1-Power_Fault 1-Flooding_Fault  1-Fire_Fault  1-Cooling_Fault  POWER]); %Operative_Level=Operative_Level*max((1-Unauthorized_Access),0.5);  Operative_Level=(1-Physical_Fault)*(1-0.5*Unauthorized_Access);, step_computed=, dynamic_computed=, step_sended=ROOM_QoS=Operative_Level;, id_entity=284, id_project=38, id_type=9, name_type=Room, color=#EDB120}
      mask prompts: Parameter1 "entity name"; Parameter2 "sampling time"; Parameter3 "project"; resources "input resources and state variables"; Parameter10 "Bring state variables to output"; codeupdate "update code from mask"
      mask help: This is a level-2 MATLAB file S-function which demonstrates CISIA entity
      mask DialogControl Container1 Prompt: All parameters
      mask Display: image('Icons/Room.png')
  Room_2 (52) : M-S-Function  FunctionName=cisia_msfun  Parameters=Parameter1, Parameter2, Parameter3, resources, Parameter10, codeupdate, step_received, step_computed, dynamic_computed, step_sended, id_entity, id_project, id_type, name_type, color  mask(S-function:msfcn_unit_delay){Parameter1='Room_2', Parameter2=1, Parameter3='ORO', resources=*** INPUT RESOURCES *** NUM_INPUTS 1 POWER (1)  *** STATE VARIABLES *** NUM_VARIABLES 8 Operative_Level(NUMERIC)(1)(1) Power_Fault(NUMERIC)(1)(0) Cooling_Fault(NUMERIC)(1)(0) Flooding_Fault(NUMERIC)(1)(0) Fire_Fault(NUMERIC)(1)(0) Unauthorized_Access(NUMERIC)(1)(0) Earthquake_Fault(NUMERIC)(1)(0) Physical_Fault(NUMERIC)(1)(0)  *** OUTPUT RESOURCES *** NUM_OUTPUTS 1 ROOM_QoS (1), Parameter10=off, codeupdate=off, step_received=Physical_Fault=max([Power_Fault Flooding_Fault Fire_Fault Cooling_Fault 1-POWER]);   %Operative_Level=min([1-Power_Fault 1-Flooding_Fault  1-Fire_Fault  1-Cooling_Fault  POWER]); %Operative_Level=Operative_Level*max((1-Unauthorized_Access),0.5);  Operative_Level=(1-Physical_Fault)*(1-0.5*Unauthorized_Access);, step_computed=, dynamic_computed=, step_sended=ROOM_QoS=Operative_Level;, id_entity=52, id_project=38, id_type=9, name_type=Room, color=#EDB120}
      mask prompts: Parameter1 "entity name"; Parameter2 "sampling time"; Parameter3 "project"; resources "input resources and state variables"; Parameter10 "Bring state variables to output"; codeupdate "update code from mask"
      mask help: This is a level-2 MATLAB file S-function which demonstrates CISIA entity
      mask DialogControl Container1 Prompt: All parameters
      mask Display: image('Icons/Room.png')
  Room_3 (200) : M-S-Function  FunctionName=cisia_msfun  Parameters=Parameter1, Parameter2, Parameter3, resources, Parameter10, codeupdate, step_received, step_computed, dynamic_computed, step_sended, id_entity, id_project, id_type, name_type, color  mask(S-function:msfcn_unit_delay){Parameter1='Room_3', Parameter2=1, Parameter3='ORO', resources=*** INPUT RESOURCES *** NUM_INPUTS 1 POWER (1)  *** STATE VARIABLES *** NUM_VARIABLES 8 Operative_Level(NUMERIC)(1)(1) Power_Fault(NUMERIC)(1)(0) Cooling_Fault(NUMERIC)(1)(0) Flooding_Fault(NUMERIC)(1)(0) Fire_Fault(NUMERIC)(1)(0) Unauthorized_Access(NUMERIC)(1)(0) Earthquake_Fault(NUMERIC)(1)(0) Physical_Fault(NUMERIC)(1)(0)  *** OUTPUT RESOURCES *** NUM_OUTPUTS 1 ROOM_QoS (1), Parameter10=off, codeupdate=off, step_received=Physical_Fault=max([Power_Fault Flooding_Fault Fire_Fault Cooling_Fault 1-POWER]);   %Operative_Level=min([1-Power_Fault 1-Flooding_Fault  1-Fire_Fault  1-Cooling_Fault  POWER]); %Operative_Level=Operative_Level*max((1-Unauthorized_Access),0.5);  Operative_Level=(1-Physical_Fault)*(1-0.5*Unauthorized_Access);, step_computed=, dynamic_computed=, step_sended=ROOM_QoS=Operative_Level;, id_entity=200, id_project=38, id_type=9, name_type=Room, color=#EDB120}
      mask prompts: Parameter1 "entity name"; Parameter2 "sampling time"; Parameter3 "project"; resources "input resources and state variables"; Parameter10 "Bring state variables to output"; codeupdate "update code from mask"
      mask help: This is a level-2 MATLAB file S-function which demonstrates CISIA entity
      mask DialogControl Container1 Prompt: All parameters
      mask Display: image('Icons/Room.png')
  Room_4 (237) : M-S-Function  FunctionName=cisia_msfun  Parameters=Parameter1, Parameter2, Parameter3, resources, Parameter10, codeupdate, step_received, step_computed, dynamic_computed, step_sended, id_entity, id_project, id_type, name_type, color  mask(S-function:msfcn_unit_delay){Parameter1='Room_4', Parameter2=1, Parameter3='ORO', resources=*** INPUT RESOURCES *** NUM_INPUTS 1 POWER (1)  *** STATE VARIABLES *** NUM_VARIABLES 8 Operative_Level(NUMERIC)(1)(1) Power_Fault(NUMERIC)(1)(0) Cooling_Fault(NUMERIC)(1)(0) Flooding_Fault(NUMERIC)(1)(0) Fire_Fault(NUMERIC)(1)(0) Unauthorized_Access(NUMERIC)(1)(0) Earthquake_Fault(NUMERIC)(1)(0) Physical_Fault(NUMERIC)(1)(0)  *** OUTPUT RESOURCES *** NUM_OUTPUTS 1 ROOM_QoS (1), Parameter10=off, codeupdate=off, step_received=Physical_Fault=max([Power_Fault Flooding_Fault Fire_Fault Cooling_Fault 1-POWER]);   %Operative_Level=min([1-Power_Fault 1-Flooding_Fault  1-Fire_Fault  1-Cooling_Fault  POWER]); %Operative_Level=Operative_Level*max((1-Unauthorized_Access),0.5);  Operative_Level=(1-Physical_Fault)*(1-0.5*Unauthorized_Access);, step_computed=, dynamic_computed=, step_sended=ROOM_QoS=Operative_Level;, id_entity=237, id_project=38, id_type=9, name_type=Room, color=#EDB120}
      mask prompts: Parameter1 "entity name"; Parameter2 "sampling time"; Parameter3 "project"; resources "input resources and state variables"; Parameter10 "Bring state variables to output"; codeupdate "update code from mask"
      mask help: This is a level-2 MATLAB file S-function which demonstrates CISIA entity
      mask DialogControl Container1 Prompt: All parameters
      mask Display: image('Icons/Room.png')
  Room_5 (240) : M-S-Function  FunctionName=cisia_msfun  Parameters=Parameter1, Parameter2, Parameter3, resources, Parameter10, codeupdate, step_received, step_computed, dynamic_computed, step_sended, id_entity, id_project, id_type, name_type, color  mask(S-function:msfcn_unit_delay){Parameter1='Room_5', Parameter2=1, Parameter3='ORO', resources=*** INPUT RESOURCES *** NUM_INPUTS 1 POWER (1)  *** STATE VARIABLES *** NUM_VARIABLES 8 Operative_Level(NUMERIC)(1)(1) Power_Fault(NUMERIC)(1)(0) Cooling_Fault(NUMERIC)(1)(0) Flooding_Fault(NUMERIC)(1)(0) Fire_Fault(NUMERIC)(1)(0) Unauthorized_Access(NUMERIC)(1)(0) Earthquake_Fault(NUMERIC)(1)(0) Physical_Fault(NUMERIC)(1)(0)  *** OUTPUT RESOURCES *** NUM_OUTPUTS 1 ROOM_QoS (1), Parameter10=off, codeupdate=off, step_received=Physical_Fault=max([Power_Fault Flooding_Fault Fire_Fault Cooling_Fault 1-POWER]);   %Operative_Level=min([1-Power_Fault 1-Flooding_Fault  1-Fire_Fault  1-Cooling_Fault  POWER]); %Operative_Level=Operative_Level*max((1-Unauthorized_Access),0.5);  Operative_Level=(1-Physical_Fault)*(1-0.5*Unauthorized_Access);, step_computed=, dynamic_computed=, step_sended=ROOM_QoS=Operative_Level;, id_entity=240, id_project=38, id_type=9, name_type=Room, color=#EDB120}
      mask prompts: Parameter1 "entity name"; Parameter2 "sampling time"; Parameter3 "project"; resources "input resources and state variables"; Parameter10 "Bring state variables to output"; codeupdate "update code from mask"
      mask help: This is a level-2 MATLAB file S-function which demonstrates CISIA entity
      mask DialogControl Container1 Prompt: All parameters
      mask Display: image('Icons/Room.png')
  Room_6 (241) : M-S-Function  FunctionName=cisia_msfun  Parameters=Parameter1, Parameter2, Parameter3, resources, Parameter10, codeupdate, step_received, step_computed, dynamic_computed, step_sended, id_entity, id_project, id_type, name_type, color  mask(S-function:msfcn_unit_delay){Parameter1='Room_6', Parameter2=1, Parameter3='ORO', resources=*** INPUT RESOURCES *** NUM_INPUTS 1 POWER (1)  *** STATE VARIABLES *** NUM_VARIABLES 8 Operative_Level(NUMERIC)(1)(1) Power_Fault(NUMERIC)(1)(0) Cooling_Fault(NUMERIC)(1)(0) Flooding_Fault(NUMERIC)(1)(0) Fire_Fault(NUMERIC)(1)(0) Unauthorized_Access(NUMERIC)(1)(0) Earthquake_Fault(NUMERIC)(1)(0) Physical_Fault(NUMERIC)(1)(0)  *** OUTPUT RESOURCES *** NUM_OUTPUTS 1 ROOM_QoS (1), Parameter10=off, codeupdate=off, step_received=Physical_Fault=max([Power_Fault Flooding_Fault Fire_Fault Cooling_Fault 1-POWER]);   %Operative_Level=min([1-Power_Fault 1-Flooding_Fault  1-Fire_Fault  1-Cooling_Fault  POWER]); %Operative_Level=Operative_Level*max((1-Unauthorized_Access),0.5);  Operative_Level=(1-Physical_Fault)*(1-0.5*Unauthorized_Access);, step_computed=, dynamic_computed=, step_sended=ROOM_QoS=Operative_Level;, id_entity=241, id_project=38, id_type=9, name_type=Room, color=#EDB120}
      mask prompts: Parameter1 "entity name"; Parameter2 "sampling time"; Parameter3 "project"; resources "input resources and state variables"; Parameter10 "Bring state variables to output"; codeupdate "update code from mask"
      mask help: This is a level-2 MATLAB file S-function which demonstrates CISIA entity
      mask DialogControl Container1 Prompt: All parameters
      mask Display: image('Icons/Room.png')
  Room_7 (252) : M-S-Function  FunctionName=cisia_msfun  Parameters=Parameter1, Parameter2, Parameter3, resources, Parameter10, codeupdate, step_received, step_computed, dynamic_computed, step_sended, id_entity, id_project, id_type, name_type, color  mask(S-function:msfcn_unit_delay){Parameter1='Room_7', Parameter2=1, Parameter3='ORO', resources=*** INPUT RESOURCES *** NUM_INPUTS 1 POWER (1)  *** STATE VARIABLES *** NUM_VARIABLES 8 Operative_Level(NUMERIC)(1)(1) Power_Fault(NUMERIC)(1)(0) Cooling_Fault(NUMERIC)(1)(0) Flooding_Fault(NUMERIC)(1)(0) Fire_Fault(NUMERIC)(1)(0) Unauthorized_Access(NUMERIC)(1)(0) Earthquake_Fault(NUMERIC)(1)(0) Physical_Fault(NUMERIC)(1)(0)  *** OUTPUT RESOURCES *** NUM_OUTPUTS 1 ROOM_QoS (1), Parameter10=off, codeupdate=off, step_received=Physical_Fault=max([Power_Fault Flooding_Fault Fire_Fault Cooling_Fault 1-POWER]);   %Operative_Level=min([1-Power_Fault 1-Flooding_Fault  1-Fire_Fault  1-Cooling_Fault  POWER]); %Operative_Level=Operative_Level*max((1-Unauthorized_Access),0.5);  Operative_Level=(1-Physical_Fault)*(1-0.5*Unauthorized_Access);, step_computed=, dynamic_computed=, step_sended=ROOM_QoS=Operative_Level;, id_entity=252, id_project=38, id_type=9, name_type=Room, color=#EDB120}
      mask prompts: Parameter1 "entity name"; Parameter2 "sampling time"; Parameter3 "project"; resources "input resources and state variables"; Parameter10 "Bring state variables to output"; codeupdate "update code from mask"
      mask help: This is a level-2 MATLAB file S-function which demonstrates CISIA entity
      mask DialogControl Container1 Prompt: All parameters
      mask Display: image('Icons/Room.png')
  Room_8 (283) : M-S-Function  FunctionName=cisia_msfun  Parameters=Parameter1, Parameter2, Parameter3, resources, Parameter10, codeupdate, step_received, step_computed, dynamic_computed, step_sended, id_entity, id_project, id_type, name_type, color  mask(S-function:msfcn_unit_delay){Parameter1='Room_8', Parameter2=1, Parameter3='ORO', resources=*** INPUT RESOURCES *** NUM_INPUTS 1 POWER (1)  *** STATE VARIABLES *** NUM_VARIABLES 8 Operative_Level(NUMERIC)(1)(1) Power_Fault(NUMERIC)(1)(0) Cooling_Fault(NUMERIC)(1)(0) Flooding_Fault(NUMERIC)(1)(0) Fire_Fault(NUMERIC)(1)(0) Unauthorized_Access(NUMERIC)(1)(0) Earthquake_Fault(NUMERIC)(1)(0) Physical_Fault(NUMERIC)(1)(0)  *** OUTPUT RESOURCES *** NUM_OUTPUTS 1 ROOM_QoS (1), Parameter10=off, codeupdate=off, step_received=Physical_Fault=max([Power_Fault Flooding_Fault Fire_Fault Cooling_Fault 1-POWER]);   %Operative_Level=min([1-Power_Fault 1-Flooding_Fault  1-Fire_Fault  1-Cooling_Fault  POWER]); %Operative_Level=Operative_Level*max((1-Unauthorized_Access),0.5);  Operative_Level=(1-Physical_Fault)*(1-0.5*Unauthorized_Access);, step_computed=, dynamic_computed=, step_sended=ROOM_QoS=Operative_Level;, id_entity=283, id_project=38, id_type=9, name_type=Room, color=#EDB120}
      mask prompts: Parameter1 "entity name"; Parameter2 "sampling time"; Parameter3 "project"; resources "input resources and state variables"; Parameter10 "Bring state variables to output"; codeupdate "update code from mask"
      mask help: This is a level-2 MATLAB file S-function which demonstrates CISIA entity
      mask DialogControl Container1 Prompt: All parameters
      mask Display: image('Icons/Room.png')
  Room_9 (255) : M-S-Function  FunctionName=cisia_msfun  Parameters=Parameter1, Parameter2, Parameter3, resources, Parameter10, codeupdate, step_received, step_computed, dynamic_computed, step_sended, id_entity, id_project, id_type, name_type, color  mask(S-function:msfcn_unit_delay){Parameter1='Room_9', Parameter2=1, Parameter3='ORO', resources=*** INPUT RESOURCES *** NUM_INPUTS 1 POWER (1)  *** STATE VARIABLES *** NUM_VARIABLES 8 Operative_Level(NUMERIC)(1)(1) Power_Fault(NUMERIC)(1)(0) Cooling_Fault(NUMERIC)(1)(0) Flooding_Fault(NUMERIC)(1)(0) Fire_Fault(NUMERIC)(1)(0) Unauthorized_Access(NUMERIC)(1)(0) Earthquake_Fault(NUMERIC)(1)(0) Physical_Fault(NUMERIC)(1)(0)  *** OUTPUT RESOURCES *** NUM_OUTPUTS 1 ROOM_QoS (1), Parameter10=off, codeupdate=off, step_received=Physical_Fault=max([Power_Fault Flooding_Fault Fire_Fault Cooling_Fault 1-POWER]);   %Operative_Level=min([1-Power_Fault 1-Flooding_Fault  1-Fire_Fault  1-Cooling_Fault  POWER]); %Operative_Level=Operative_Level*max((1-Unauthorized_Access),0.5);  Operative_Level=(1-Physical_Fault)*(1-0.5*Unauthorized_Access);, step_computed=, dynamic_computed=, step_sended=ROOM_QoS=Operative_Level;, id_entity=255, id_project=38, id_type=9, name_type=Room, color=#EDB120}
      mask prompts: Parameter1 "entity name"; Parameter2 "sampling time"; Parameter3 "project"; resources "input resources and state variables"; Parameter10 "Bring state variables to output"; codeupdate "update code from mask"
      mask help: This is a level-2 MATLAB file S-function which demonstrates CISIA entity
      mask DialogControl Container1 Prompt: All parameters
      mask Display: image('Icons/Room.png')
  Room_Qos12 : MinMax  Inputs=2
  SAVE_1 (1) : M-S-Function  FunctionName=cisia_msfun  Parameters=Parameter1, Parameter2, Parameter3, Parameter4,Parameter5,Parameter6,Parameter7  mask(S-function:msfcn_unit_delay){Parameter1='SAVE_1', Parameter2=1, Parameter3='SistemiIoT', Parameter4=on, Parameter5=[1], Parameter6=[1], Parameter7=off}
      mask prompts: Parameter1 "entity name"; Parameter2 "sampling time"; Parameter3 "project"; Parameter4 "display bars"; Parameter5 "values"; Parameter6 "logic"; Parameter7 "display B/W"
      mask help: This is a level-2 MATLAB file S-function which demonstrates CISIA entity
      mask DialogControl Container3 Prompt: Display
      mask Display: disp('SAVE')
  SAVE_13 (13) : M-S-Function  FunctionName=cisia_msfun  Parameters=Parameter1, Parameter2, Parameter3, Parameter4,Parameter5,Parameter6,Parameter7  mask(S-function:msfcn_unit_delay){Parameter1='SAVE_13', Parameter2=1, Parameter3='SistemiIoT', Parameter4=on, Parameter5=[1], Parameter6=[1], Parameter7=off}
      mask prompts: Parameter1 "entity name"; Parameter2 "sampling time"; Parameter3 "project"; Parameter4 "display bars"; Parameter5 "values"; Parameter6 "logic"; Parameter7 "display B/W"
      mask help: This is a level-2 MATLAB file S-function which demonstrates CISIA entity
      mask DialogControl Container3 Prompt: Display
      mask Display: disp('SAVE')
  SAVE_14 (14) : M-S-Function  FunctionName=cisia_msfun  Parameters=Parameter1, Parameter2, Parameter3, Parameter4,Parameter5,Parameter6,Parameter7  mask(S-function:msfcn_unit_delay){Parameter1='SAVE_14', Parameter2=1, Parameter3='SistemiIoT', Parameter4=on, Parameter5=[1], Parameter6=[1], Parameter7=off}
      mask prompts: Parameter1 "entity name"; Parameter2 "sampling time"; Parameter3 "project"; Parameter4 "display bars"; Parameter5 "values"; Parameter6 "logic"; Parameter7 "display B/W"
      mask help: This is a level-2 MATLAB file S-function which demonstrates CISIA entity
      mask DialogControl Container3 Prompt: Display
      mask Display: disp('SAVE')
  SAVE_15 (15) : M-S-Function  FunctionName=cisia_msfun  Parameters=Parameter1, Parameter2, Parameter3, Parameter4,Parameter5,Parameter6,Parameter7  mask(S-function:msfcn_unit_delay){Parameter1='SAVE_15', Parameter2=1, Parameter3='SistemiIoT', Parameter4=on, Parameter5=[1], Parameter6=[1], Parameter7=off}
      mask prompts: Parameter1 "entity name"; Parameter2 "sampling time"; Parameter3 "project"; Parameter4 "display bars"; Parameter5 "values"; Parameter6 "logic"; Parameter7 "display B/W"
      mask help: This is a level-2 MATLAB file S-function which demonstrates CISIA entity
      mask DialogControl Container3 Prompt: Display
      mask Display: disp('SAVE')
  SAVE_16 (16) : M-S-Function  FunctionName=cisia_msfun  Parameters=Parameter1, Parameter2, Parameter3, Parameter4,Parameter5,Parameter6,Parameter7  mask(S-function:msfcn_unit_delay){Parameter1='SAVE_16', Parameter2=1, Parameter3='SistemiIoT', Parameter4=on, Parameter5=[1], Parameter6=[1], Parameter7=off}
      mask prompts: Parameter1 "entity name"; Parameter2 "sampling time"; Parameter3 "project"; Parameter4 "display bars"; Parameter5 "values"; Parameter6 "logic"; Parameter7 "display B/W"
      mask help: This is a level-2 MATLAB file S-function which demonstrates CISIA entity
      mask DialogControl Container3 Prompt: Display
      mask Display: disp('SAVE')
  SAVE_17 (17) : M-S-Function  FunctionName=cisia_msfun  Parameters=Parameter1, Parameter2, Parameter3, Parameter4,Parameter5,Parameter6,Parameter7  mask(S-function:msfcn_unit_delay){Parameter1='SAVE_17', Parameter2=1, Parameter3='SistemiIoT', Parameter4=on, Parameter5=[1], Parameter6=[1], Parameter7=off}
      mask prompts: Parameter1 "entity name"; Parameter2 "sampling time"; Parameter3 "project"; Parameter4 "display bars"; Parameter5 "values"; Parameter6 "logic"; Parameter7 "display B/W"
      mask help: This is a level-2 MATLAB file S-function which demonstrates CISIA entity
      mask DialogControl Container3 Prompt: Display
      mask Display: disp('SAVE')
  SAVE_18 (18) : M-S-Function  FunctionName=cisia_msfun  Parameters=Parameter1, Parameter2, Parameter3, Parameter4,Parameter5,Parameter6,Parameter7  mask(S-function:msfcn_unit_delay){Parameter1='SAVE_18', Parameter2=1, Parameter3='SistemiIoT', Parameter4=on, Parameter5=[1], Parameter6=[1], Parameter7=off}
      mask prompts: Parameter1 "entity name"; Parameter2 "sampling time"; Parameter3 "project"; Parameter4 "display bars"; Parameter5 "values"; Parameter6 "logic"; Parameter7 "display B/W"
      mask help: This is a level-2 MATLAB file S-function which demonstrates CISIA entity
      mask DialogControl Container3 Prompt: Display
      mask Display: disp('SAVE')
  SAVE_19 (19) : M-S-Function  FunctionName=cisia_msfun  Parameters=Parameter1, Parameter2, Parameter3, Parameter4,Parameter5,Parameter6,Parameter7  mask(S-function:msfcn_unit_delay){Parameter1='SAVE_19', Parameter2=1, Parameter3='SistemiIoT', Parameter4=on, Parameter5=[1], Parameter6=[1], Parameter7=off}
      mask prompts: Parameter1 "entity name"; Parameter2 "sampling time"; Parameter3 "project"; Parameter4 "display bars"; Parameter5 "values"; Parameter6 "logic"; Parameter7 "display B/W"
      mask help: This is a level-2 MATLAB file S-function which demonstrates CISIA entity
      mask DialogControl Container3 Prompt: Display
      mask Display: disp('SAVE')
  SAVE_2 (2) : M-S-Function  FunctionName=cisia_msfun  Parameters=Parameter1, Parameter2, Parameter3, Parameter4,Parameter5,Parameter6,Parameter7  mask(S-function:msfcn_unit_delay){Parameter1='SAVE_2', Parameter2=1, Parameter3='SistemiIoT', Parameter4=on, Parameter5=[1], Parameter6=[1], Parameter7=off}
      mask prompts: Parameter1 "entity name"; Parameter2 "sampling time"; Parameter3 "project"; Parameter4 "display bars"; Parameter5 "values"; Parameter6 "logic"; Parameter7 "display B/W"
      mask help: This is a level-2 MATLAB file S-function which demonstrates CISIA entity
      mask DialogControl Container3 Prompt: Display
      mask Display: disp('SAVE')
  SAVE_20 (20) : M-S-Function  FunctionName=cisia_msfun  Parameters=Parameter1, Parameter2, Parameter3, Parameter4,Parameter5,Parameter6,Parameter7  mask(S-function:msfcn_unit_delay){Parameter1='SAVE_20', Parameter2=1, Parameter3='SistemiIoT', Parameter4=on, Parameter5=[1], Parameter6=[1], Parameter7=off}
      mask prompts: Parameter1 "entity name"; Parameter2 "sampling time"; Parameter3 "project"; Parameter4 "display bars"; Parameter5 "values"; Parameter6 "logic"; Parameter7 "display B/W"
      mask help: This is a level-2 MATLAB file S-function which demonstrates CISIA entity
      mask DialogControl Container3 Prompt: Display
      mask Display: disp('SAVE')
  SAVE_21 (21) : M-S-Function  FunctionName=cisia_msfun  Parameters=Parameter1, Parameter2, Parameter3, Parameter4,Parameter5,Parameter6,Parameter7  mask(S-function:msfcn_unit_delay){Parameter1='SAVE_21', Parameter2=1, Parameter3='SistemiIoT', Parameter4=on, Parameter5=[1], Parameter6=[1], Parameter7=off}
      mask prompts: Parameter1 "entity name"; Parameter2 "sampling time"; Parameter3 "project"; Parameter4 "display bars"; Parameter5 "values"; Parameter6 "logic"; Parameter7 "display B/W"
      mask help: This is a level-2 MATLAB file S-function which demonstrates CISIA entity
      mask DialogControl Container3 Prompt: Display
      mask Display: disp('SAVE')
  SAVE_22 (22) : M-S-Function  FunctionName=cisia_msfun  Parameters=Parameter1, Parameter2, Parameter3, Parameter4,Parameter5,Parameter6,Parameter7  mask(S-function:msfcn_unit_delay){Parameter1='SAVE_22', Parameter2=1, Parameter3='SistemiIoT', Parameter4=on, Parameter5=[1], Parameter6=[1], Parameter7=off}
      mask prompts: Parameter1 "entity name"; Parameter2 "sampling time"; Parameter3 "project"; Parameter4 "display bars"; Parameter5 "values"; Parameter6 "logic"; Parameter7 "display B/W"
      mask help: This is a level-2 MATLAB file S-function which demonstrates CISIA entity
      mask DialogControl Container3 Prompt: Display
      mask Display: disp('SAVE')
  SAVE_23 (23) : M-S-Function  FunctionName=cisia_msfun  Parameters=Parameter1, Parameter2, Parameter3, Parameter4,Parameter5,Parameter6,Parameter7  mask(S-function:msfcn_unit_delay){Parameter1='SAVE_23', Parameter2=1, Parameter3='SistemiIoT', Parameter4=on, Parameter5=[0], Parameter6=[1], Parameter7=off}
      mask prompts: Parameter1 "entity name"; Parameter2 "sampling time"; Parameter3 "project"; Parameter4 "display bars"; Parameter5 "values"; Parameter6 "logic"; Parameter7 "display B/W"
      mask help: This is a level-2 MATLAB file S-function which demonstrates CISIA entity
      mask DialogControl Container3 Prompt: Display
      mask Display: disp('SAVE')
  SAVE_3 (3) : M-S-Function  FunctionName=cisia_msfun  Parameters=Parameter1, Parameter2, Parameter3, Parameter4,Parameter5,Parameter6,Parameter7  mask(S-function:msfcn_unit_delay){Parameter1='SAVE_3', Parameter2=1, Parameter3='SistemiIoT', Parameter4=on, Parameter5=[1], Parameter6=[1], Parameter7=off}
      mask prompts: Parameter1 "entity name"; Parameter2 "sampling time"; Parameter3 "project"; Parameter4 "display bars"; Parameter5 "values"; Parameter6 "logic"; Parameter7 "display B/W"
      mask help: This is a level-2 MATLAB file S-function which demonstrates CISIA entity
      mask DialogControl Container3 Prompt: Display
      mask Display: disp('SAVE')
  SAVE_4 (4) : M-S-Function  FunctionName=cisia_msfun  Parameters=Parameter1, Parameter2, Parameter3, Parameter4,Parameter5,Parameter6,Parameter7  mask(S-function:msfcn_unit_delay){Parameter1='SAVE_4', Parameter2=1, Parameter3='SistemiIoT', Parameter4=on, Parameter5=[1], Parameter6=[1], Parameter7=off}
      mask prompts: Parameter1 "entity name"; Parameter2 "sampling time"; Parameter3 "project"; Parameter4 "display bars"; Parameter5 "values"; Parameter6 "logic"; Parameter7 "display B/W"
      mask help: This is a level-2 MATLAB file S-function which demonstrates CISIA entity
      mask DialogControl Container3 Prompt: Display
      mask Display: disp('SAVE')
  SAVE_5 (5) : M-S-Function  FunctionName=cisia_msfun  Parameters=Parameter1, Parameter2, Parameter3, Parameter4,Parameter5,Parameter6,Parameter7  mask(S-function:msfcn_unit_delay){Parameter1='SAVE_5', Parameter2=1, Parameter3='SistemiIoT', Parameter4=on, Parameter5=[1], Parameter6=[1], Parameter7=off}
      mask prompts: Parameter1 "entity name"; Parameter2 "sampling time"; Parameter3 "project"; Parameter4 "display bars"; Parameter5 "values"; Parameter6 "logic"; Parameter7 "display B/W"
      mask help: This is a level-2 MATLAB file S-function which demonstrates CISIA entity
      mask DialogControl Container3 Prompt: Display
      mask Display: disp('SAVE')
  SAVE_6 (6) : M-S-Function  FunctionName=cisia_msfun  Parameters=Parameter1, Parameter2, Parameter3, Parameter4,Parameter5,Parameter6,Parameter7  mask(S-function:msfcn_unit_delay){Parameter1='SAVE_6', Parameter2=1, Parameter3='SistemiIoT', Parameter4=on, Parameter5=[1], Parameter6=[1], Parameter7=off}
      mask prompts: Parameter1 "entity name"; Parameter2 "sampling time"; Parameter3 "project"; Parameter4 "display bars"; Parameter5 "values"; Parameter6 "logic"; Parameter7 "display B/W"
      mask help: This is a level-2 MATLAB file S-function which demonstrates CISIA entity
      mask DialogControl Container3 Prompt: Display
      mask Display: disp('SAVE')
  SAVE_7 (7) : M-S-Function  FunctionName=cisia_msfun  Parameters=Parameter1, Parameter2, Parameter3, Parameter4,Parameter5,Parameter6,Parameter7  mask(S-function:msfcn_unit_delay){Parameter1='SAVE_7', Parameter2=1, Parameter3='SistemiIoT', Parameter4=on, Parameter5=[1], Parameter6=[1], Parameter7=off}
      mask prompts: Parameter1 "entity name"; Parameter2 "sampling time"; Parameter3 "project"; Parameter4 "display bars"; Parameter5 "values"; Parameter6 "logic"; Parameter7 "display B/W"
      mask help: This is a level-2 MATLAB file S-function which demonstrates CISIA entity
      mask DialogControl Container3 Prompt: Display
      mask Display: disp('SAVE')
  SAVE_8 (8) : M-S-Function  FunctionName=cisia_msfun  Parameters=Parameter1, Parameter2, Parameter3, Parameter4,Parameter5,Parameter6,Parameter7  mask(S-function:msfcn_unit_delay){Parameter1='SAVE_8', Parameter2=1, Parameter3='SistemiIoT', Parameter4=on, Parameter5=[1], Parameter6=[1], Parameter7=off}
      mask prompts: Parameter1 "entity name"; Parameter2 "sampling time"; Parameter3 "project"; Parameter4 "display bars"; Parameter5 "values"; Parameter6 "logic"; Parameter7 "display B/W"
      mask help: This is a level-2 MATLAB file S-function which demonstrates CISIA entity
      mask DialogControl Container3 Prompt: Display
      mask Display: disp('SAVE')
  SAVE_9 (9) : M-S-Function  FunctionName=cisia_msfun  Parameters=Parameter1, Parameter2, Parameter3, Parameter4,Parameter5,Parameter6,Parameter7  mask(S-function:msfcn_unit_delay){Parameter1='SAVE_9', Parameter2=1, Parameter3='SistemiIoT', Parameter4=on, Parameter5=[1], Parameter6=[1], Parameter7=off}
      mask prompts: Parameter1 "entity name"; Parameter2 "sampling time"; Parameter3 "project"; Parameter4 "display bars"; Parameter5 "values"; Parameter6 "logic"; Parameter7 "display B/W"
      mask help: This is a level-2 MATLAB file S-function which demonstrates CISIA entity
      mask DialogControl Container3 Prompt: Display
      mask Display: disp('SAVE')
  Splitter_1 (54) : M-S-Function  FunctionName=cisia_msfun  Parameters=Parameter1, Parameter2, Parameter3, resources, Parameter10, codeupdate, step_received, step_computed, dynamic_computed, step_sended, id_entity, id_project, id_type, name_type, color  mask(S-function:msfcn_unit_delay){Parameter1='Splitter_1', Parameter2=1, Parameter3='ORO', resources=*** INPUT RESOURCES *** NUM_INPUTS 3 TLC_SERVICE (20) CYBER_FAULT (10) NGPON_CONN (20)  *** STATE VARIABLES *** NUM_VARIABLES 18 Operative_Level(NUMERIC)(1)(1) TLC_services(NUMERIC_ARRAY)(20)(0  0  0  0  0  0  0  0  0  0  0  0  0  0  0  0  0  0  0  0) Connection(NUMERIC_ARRAY)(20)(0  0  0  0  0  0  0  0  0  0  0  0  0  0  0  0  0  0  0  0) Dos_attack(NUMERIC)(1)(0) MITM_attack(NUMERIC)(1)(0) Virus_Attack(NUMERIC)(1)(0) Port_Scan_Attack(NUMERIC)(1)(0) Cyber_Fault(NUMERIC_ARRAY)(10)(0  0  0  0  0  0  0  0  0  0) MyConn(NUMERIC_ARRAY)(20)(0  0  0  0  0  0  0  0  0  0  0  0  0  0  0  0  0  0  0  0) BGP_hijacking(NUMERIC)(1)(0) Mechanical_Fault(NUMERIC)(1)(0) Conn_Fault(NUMERIC)(1)(0) BotNet_Attack(NUMERIC)(1)(0) Data_Corruption(NUMERIC)(1)(0) SW_Change(NUMERIC)(1)(0) Config_Change(NUMERIC)(1)(0) Port_Saturation(NUMERIC)(1)(0) TLC_revoke(NUMERIC_ARRAY)(20)(0  0  0  0  0  0  0  0  0  0  0  0  0  0  0  0  0  0  0  0)  *** OUTPUT RESOURCES *** NUM_OUTPUTS 4 TLC_SERVICE (20) CYBER_FAULT (10) NGPON_CONN (20) NGPON_IN (20), Parameter10=off, codeupdate=off, step_received=Connection=max(Connection_init,NGPON_CONN); TLC_services=max(TLC_services_init,TLC_SERVICE); TLC_services=mod(TLC_services,10); TLC_revoke=floor(TLC_SERVICE/10);  Cyber_Fault=max(CYBER_FAULT, transpose([Dos_attack   MITM_attack Virus_Attack Port_Scan_Attack  BGP_hijacking BotNet_Attack Data_Corruption SW_Change Config_Change Port_Saturation]));  % Vale 1 in presenza di fault Conn_Fault=max([Dos_attack  Mechanical_Fault] );  Operative_Level=(1-Conn_Fault)*max(max(NGPON_CONN),0.5)*(1-0.5*max(Cyber_Fault)) ;, step_computed=, dynamic_computed=, step_sended=NGPON_IN=Connection;  NGPON_CONN=Connection*(1-Conn_Fault); TLC_SERVICE=TLC_services*(1-Conn_Fault)+10*TLC_revoke;  Cyber_Transmitted=min(Cyber_Fault, transpose([0 0 1 0 1 1 0 0 0 1])); CYBER_FAULT=Cyber_Transmitted*(1-Conn_Fault);   ROUTING_QoS=Operative_Level;, id_entity=54, id_project=38, id_type=11, name_type=Splitter, color=#90DB5A}
      mask prompts: Parameter1 "entity name"; Parameter2 "sampling time"; Parameter3 "project"; resources "input resources and state variables"; Parameter10 "Bring state variables to output"; codeupdate "update code from mask"
      mask help: This is a level-2 MATLAB file S-function which demonstrates CISIA entity
      mask DialogControl Container1 Prompt: All parameters
      mask Display: disp('Splitter')
  Staff_Room (183) : M-S-Function  FunctionName=cisia_msfun  Parameters=Parameter1, Parameter2, Parameter3, resources, Parameter10, codeupdate, step_received, step_computed, dynamic_computed, step_sended, id_entity, id_project, id_type, name_type, color  mask(S-function:msfcn_unit_delay){Parameter1='Staff_Room', Parameter2=1, Parameter3='ORO', resources=*** INPUT RESOURCES *** NUM_INPUTS 2 POWER (1) AIR (1)  *** STATE VARIABLES *** NUM_VARIABLES 4 Operative_Level(NUMERIC)(1)(1) Power_Fault(NUMERIC)(1)(0) Fire_Fault(NUMERIC)(1)(0) Air_Fault(NUMERIC)(1)(0)  *** OUTPUT RESOURCES *** NUM_OUTPUTS 1 ORDINARY_ROOM_QoS (1), Parameter10=off, codeupdate=off, step_received=Power_Fault=1-POWER; Air_Fault=1-AIR;   Operative_Level=(1-Fire_Fault)*(1-0.5*Power_Fault)*(1-0-5*Air_Fault);, step_computed=, dynamic_computed=, step_sended=ORDINARY_ROOM_QoS= Operative_Level;, id_entity=183, id_project=38, id_type=26, name_type=Ordinary_Room, color=#FFFFFF}
      mask prompts: Parameter1 "entity name"; Parameter2 "sampling time"; Parameter3 "project"; resources "input resources and state variables"; Parameter10 "Bring state variables to output"; codeupdate "update code from mask"
      mask help: This is a level-2 MATLAB file S-function which demonstrates CISIA entity
      mask DialogControl Container1 Prompt: All parameters
      mask Display: disp('Ordinary_Room')
  Subsystem12 : Subsystem
  Surgery (179) : M-S-Function  FunctionName=cisia_msfun  Parameters=Parameter1, Parameter2, Parameter3, resources, Parameter10, codeupdate, step_received, step_computed, dynamic_computed, step_sended, id_entity, id_project, id_type, name_type, color  mask(S-function:msfcn_unit_delay){Parameter1='Surgery', Parameter2=1, Parameter3='ORO', resources=*** INPUT RESOURCES *** NUM_INPUTS 2 POWER (1) AIR (1)  *** STATE VARIABLES *** NUM_VARIABLES 4 Operative_Level(NUMERIC)(1)(1) Power_Fault(NUMERIC)(1)(0) Fire_Fault(NUMERIC)(1)(0) Air_Fault(NUMERIC)(1)(0)  *** OUTPUT RESOURCES *** NUM_OUTPUTS 1 ORDINARY_ROOM_QoS (1), Parameter10=off, codeupdate=off, step_received=Power_Fault=1-POWER; Air_Fault=1-AIR;   Operative_Level=(1-Fire_Fault)*(1-0.5*Power_Fault)*(1-0-5*Air_Fault);, step_computed=, dynamic_computed=, step_sended=ORDINARY_ROOM_QoS= Operative_Level;, id_entity=179, id_project=38, id_type=26, name_type=Ordinary_Room, color=#FFFFFF}
      mask prompts: Parameter1 "entity name"; Parameter2 "sampling time"; Parameter3 "project"; resources "input resources and state variables"; Parameter10 "Bring state variables to output"; codeupdate "update code from mask"
      mask help: This is a level-2 MATLAB file S-function which demonstrates CISIA entity
      mask DialogControl Container1 Prompt: All parameters
      mask Display: disp('Ordinary_Room')
  TLC_conn{1..6,9} (7 alike) : MinMax  Function=max  Inputs=3
  TLC_conn{10,13..15} (4 alike) : MinMax  Function=max  Inputs=2
  TLC_conn11 : MinMax  Function=max  Inputs=4
  TLC_conn8 : MinMax  Function=max  Inputs=4
  TLC_service{1..6,9} (7 alike) : MinMax  Function=max  Inputs=3
  TLC_service{10..12,14} (4 alike) : MinMax  Function=max  Inputs=2
  TLC_service13 : MinMax  Function=max  Inputs=4
  TLC_service8 : MinMax  Function=max  Inputs=4
  Tap (119) : M-S-Function  FunctionName=cisia_msfun  Parameters=Parameter1, Parameter2, Parameter3, resources, Parameter10, codeupdate, step_received, step_computed, dynamic_computed, step_sended, id_entity, id_project, id_type, name_type, color  mask(S-function:msfcn_unit_delay){Parameter1='Tap', Parameter2=1, Parameter3='ORO', resources=*** INPUT RESOURCES *** NUM_INPUTS 0  *** STATE VARIABLES *** NUM_VARIABLES 2 Operative_Level(NUMERIC)(1)(1) Mechanical_Fault(NUMERIC)(1)(0)  *** OUTPUT RESOURCES *** NUM_OUTPUTS 1 WATER (1), Parameter10=off, codeupdate=off, step_received=Operative_Level=1-Mechanical_Fault;, step_computed=, dynamic_computed=, step_sended=WATER=1-Mechanical_Fault;, id_entity=119, id_project=38, id_type=30, name_type=Tap, color=#FFFFFF}
      mask prompts: Parameter1 "entity name"; Parameter2 "sampling time"; Parameter3 "project"; resources "input resources and state variables"; Parameter10 "Bring state variables to output"; codeupdate "update code from mask"
      mask help: This is a level-2 MATLAB file S-function which demonstrates CISIA entity
      mask DialogControl Container1 Prompt: All parameters
      mask Display: disp('Tap')
  Terminator : Terminator
  Terminator5 : Terminator
  Visit_Room (184) : M-S-Function  FunctionName=cisia_msfun  Parameters=Parameter1, Parameter2, Parameter3, resources, Parameter10, codeupdate, step_received, step_computed, dynamic_computed, step_sended, id_entity, id_project, id_type, name_type, color  mask(S-function:msfcn_unit_delay){Parameter1='Visit_Room', Parameter2=1, Parameter3='ORO', resources=*** INPUT RESOURCES *** NUM_INPUTS 2 POWER (1) AIR (1)  *** STATE VARIABLES *** NUM_VARIABLES 4 Operative_Level(NUMERIC)(1)(1) Power_Fault(NUMERIC)(1)(0) Fire_Fault(NUMERIC)(1)(0) Air_Fault(NUMERIC)(1)(0)  *** OUTPUT RESOURCES *** NUM_OUTPUTS 1 ORDINARY_ROOM_QoS (1), Parameter10=off, codeupdate=off, step_received=Power_Fault=1-POWER; Air_Fault=1-AIR;   Operative_Level=(1-Fire_Fault)*(1-0.5*Power_Fault)*(1-0-5*Air_Fault);, step_computed=, dynamic_computed=, step_sended=ORDINARY_ROOM_QoS= Operative_Level;, id_entity=184, id_project=38, id_type=26, name_type=Ordinary_Room, color=#FFFFFF}
      mask prompts: Parameter1 "entity name"; Parameter2 "sampling time"; Parameter3 "project"; resources "input resources and state variables"; Parameter10 "Bring state variables to output"; codeupdate "update code from mask"
      mask help: This is a level-2 MATLAB file S-function which demonstrates CISIA entity
      mask DialogControl Container1 Prompt: All parameters
      mask Display: disp('Ordinary_Room')
  WS : MinMax  Inputs=2
  Waiting_Room (180) : M-S-Function  FunctionName=cisia_msfun  Parameters=Parameter1, Parameter2, Parameter3, resources, Parameter10, codeupdate, step_received, step_computed, dynamic_computed, step_sended, id_entity, id_project, id_type, name_type, color  mask(S-function:msfcn_unit_delay){Parameter1='Waiting_Room', Parameter2=1, Parameter3='ORO', resources=*** INPUT RESOURCES *** NUM_INPUTS 2 POWER (1) AIR (1)  *** STATE VARIABLES *** NUM_VARIABLES 4 Operative_Level(NUMERIC)(1)(1) Power_Fault(NUMERIC)(1)(0) Fire_Fault(NUMERIC)(1)(0) Air_Fault(NUMERIC)(1)(0)  *** OUTPUT RESOURCES *** NUM_OUTPUTS 1 ORDINARY_ROOM_QoS (1), Parameter10=off, codeupdate=off, step_received=Power_Fault=1-POWER; Air_Fault=1-AIR;   Operative_Level=(1-Fire_Fault)*(1-0.5*Power_Fault)*(1-0-5*Air_Fault);, step_computed=, dynamic_computed=, step_sended=ORDINARY_ROOM_QoS= Operative_Level;, id_entity=180, id_project=38, id_type=26, name_type=Ordinary_Room, color=#FFFFFF}
      mask prompts: Parameter1 "entity name"; Parameter2 "sampling time"; Parameter3 "project"; resources "input resources and state variables"; Parameter10 "Bring state variables to output"; codeupdate "update code from mask"
      mask help: This is a level-2 MATLAB file S-function which demonstrates CISIA entity
      mask DialogControl Container1 Prompt: All parameters
      mask Display: disp('Ordinary_Room')
  Wire_1 (1) : M-S-Function  FunctionName=cisia_msfun  Parameters=Parameter1, Parameter2, Parameter3, resources, Parameter10, codeupdate, step_received, step_computed, dynamic_computed, step_sended, id_entity, id_project, id_type, name_type, color  mask(S-function:msfcn_unit_delay){Parameter1='Wire_1', Parameter2=1, Parameter3='ORO', resources=*** INPUT RESOURCES *** NUM_INPUTS 4 TLC_CONN (20) TLC_SERVICE (20) CYBER_FAULT (10) MECH_FAULT (1)  *** STATE VARIABLES *** NUM_VARIABLES 11 Operative_Level(NUMERIC)(1)(1) TLC_services(NUMERIC_ARRAY)(20)(0  0  0  0  0  0  0  0  0  0  0  0  0  0  0  0  0  0  0  0) Connection(NUMERIC_ARRAY)(20)(0  0  0  0  0  0  0  0  0  0  0  0  0  0  0  0  0  0  0  0) Dos_attack(NUMERIC)(1)(0) MITM_attack(NUMERIC)(1)(0) Virus_Attack(NUMERIC)(1)(0) Port_Scan_Attack(NUMERIC)(1)(0) Cyber_Fault(NUMERIC_ARRAY)(10)(0  0  0  0  0  0  0  0  0  0) Mechanical_Fault(NUMERIC)(1)(0) Conn_Fault(NUMERIC)(1)(0) TLC_revoke(NUMERIC_ARRAY)(20)(0  0  0  0  0  0  0  0  0  0  0  0  0  0  0  0  0  0  0  0)  *** OUTPUT RESOURCES *** NUM_OUTPUTS 4 TLC_CONN (20) TLC_SERVICE (20) CYBER_FAULT (10) MECH_FAULT (1), Parameter10=off, codeupdate=off, step_received=Connection=max(Connection_init,TLC_CONN); TLC_services=max(TLC_services_init,TLC_SERVICE); TLC_services=mod(TLC_services,10); TLC_revoke=floor(TLC_SERVICE/10);  Cyber_Fault=CYBER_FAULT;  Mechanical_Fault=max([Mechanical_Fault MECH_FAULT Mechanical_Fault_init]);  %TLC_services=TLC_services.*(1-TLC_revoke);  Operative_Level=1-Mechanical_Fault;, step_computed=, dynamic_computed=, step_sended=TLC_CONN=Connection*Operative_Level; TLC_SERVICE=TLC_services*Operative_Level+TLC_revoke*10;   CYBER_FAULT=Cyber_Fault*Operative_Level; MECH_FAULT=Mechanical_Fault;, id_entity=1, id_project=38, id_type=1, name_type=Optical_Wire, color=#99CCFF}
      mask prompts: Parameter1 "entity name"; Parameter2 "sampling time"; Parameter3 "project"; resources "input resources and state variables"; Parameter10 "Bring state variables to output"; codeupdate "update code from mask"
      mask help: This is a level-2 MATLAB file S-function which demonstrates CISIA entity
      mask DialogControl Container1 Prompt: All parameters
      mask Display: image('Icons/Optical_Wire.png')
  Wire_10 (30) : M-S-Function  FunctionName=cisia_msfun  Parameters=Parameter1, Parameter2, Parameter3, resources, Parameter10, codeupdate, step_received, step_computed, dynamic_computed, step_sended, id_entity, id_project, id_type, name_type, color  mask(S-function:msfcn_unit_delay){Parameter1='Wire_10', Parameter2=1, Parameter3='ORO', resources=*** INPUT RESOURCES *** NUM_INPUTS 4 TLC_CONN (20) TLC_SERVICE (20) CYBER_FAULT (10) MECH_FAULT (1)  *** STATE VARIABLES *** NUM_VARIABLES 11 Operative_Level(NUMERIC)(1)(1) TLC_services(NUMERIC_ARRAY)(20)(0  0  0  0  0  0  0  0  0  0  0  0  0  0  0  0  0  0  0  0) Connection(NUMERIC_ARRAY)(20)(0  0  0  0  0  0  0  0  0  0  0  0  0  0  0  0  0  0  0  0) Dos_attack(NUMERIC)(1)(0) MITM_attack(NUMERIC)(1)(0) Virus_Attack(NUMERIC)(1)(0) Port_Scan_Attack(NUMERIC)(1)(0) Cyber_Fault(NUMERIC_ARRAY)(10)(0  0  0  0  0  0  0  0  0  0) Mechanical_Fault(NUMERIC)(1)(0) Conn_Fault(NUMERIC)(1)(0) TLC_revoke(NUMERIC_ARRAY)(20)(0  0  0  0  0  0  0  0  0  0  0  0  0  0  0  0  0  0  0  0)  *** OUTPUT RESOURCES *** NUM_OUTPUTS 4 TLC_CONN (20) TLC_SERVICE (20) CYBER_FAULT (10) MECH_FAULT (1), Parameter10=off, codeupdate=off, step_received=Connection=max(Connection_init,TLC_CONN); TLC_services=max(TLC_services_init,TLC_SERVICE); TLC_services=mod(TLC_services,10); TLC_revoke=floor(TLC_SERVICE/10);  Cyber_Fault=CYBER_FAULT;  Mechanical_Fault=max([Mechanical_Fault MECH_FAULT Mechanical_Fault_init]);  %TLC_services=TLC_services.*(1-TLC_revoke);  Operative_Level=1-Mechanical_Fault;, step_computed=, dynamic_computed=, step_sended=TLC_CONN=Connection*Operative_Level; TLC_SERVICE=TLC_services*Operative_Level+TLC_revoke*10;   CYBER_FAULT=Cyber_Fault*Operative_Level; MECH_FAULT=Mechanical_Fault;, id_entity=30, id_project=38, id_type=1, name_type=Optical_Wire, color=#99CCFF}
      mask prompts: Parameter1 "entity name"; Parameter2 "sampling time"; Parameter3 "project"; resources "input resources and state variables"; Parameter10 "Bring state variables to output"; codeupdate "update code from mask"
      mask help: This is a level-2 MATLAB file S-function which demonstrates CISIA entity
      mask DialogControl Container1 Prompt: All parameters
      mask Display: image('Icons/Optical_Wire.png')
  Wire_10b (31) : M-S-Function  FunctionName=cisia_msfun  Parameters=Parameter1, Parameter2, Parameter3, resources, Parameter10, codeupdate, step_received, step_computed, dynamic_computed, step_sended, id_entity, id_project, id_type, name_type, color  mask(S-function:msfcn_unit_delay){Parameter1='Wire_10b', Parameter2=1, Parameter3='ORO', resources=*** INPUT RESOURCES *** NUM_INPUTS 4 TLC_CONN (20) TLC_SERVICE (20) CYBER_FAULT (10) MECH_FAULT (1)  *** STATE VARIABLES *** NUM_VARIABLES 11 Operative_Level(NUMERIC)(1)(1) TLC_services(NUMERIC_ARRAY)(20)(0  0  0  0  0  0  0  0  0  0  0  0  0  0  0  0  0  0  0  0) Connection(NUMERIC_ARRAY)(20)(0  0  0  0  0  0  0  0  0  0  0  0  0  0  0  0  0  0  0  0) Dos_attack(NUMERIC)(1)(0) MITM_attack(NUMERIC)(1)(0) Virus_Attack(NUMERIC)(1)(0) Port_Scan_Attack(NUMERIC)(1)(0) Cyber_Fault(NUMERIC_ARRAY)(10)(0  0  0  0  0  0  0  0  0  0) Mechanical_Fault(NUMERIC)(1)(0) Conn_Fault(NUMERIC)(1)(0) TLC_revoke(NUMERIC_ARRAY)(20)(0  0  0  0  0  0  0  0  0  0  0  0  0  0  0  0  0  0  0  0)  *** OUTPUT RESOURCES *** NUM_OUTPUTS 4 TLC_CONN (20) TLC_SERVICE (20) CYBER_FAULT (10) MECH_FAULT (1), Parameter10=off, codeupdate=off, step_received=Connection=max(Connection_init,TLC_CONN); TLC_services=max(TLC_services_init,TLC_SERVICE); TLC_services=mod(TLC_services,10); TLC_revoke=floor(TLC_SERVICE/10);  Cyber_Fault=CYBER_FAULT;  Mechanical_Fault=max([Mechanical_Fault MECH_FAULT Mechanical_Fault_init]);  %TLC_services=TLC_services.*(1-TLC_revoke);  Operative_Level=1-Mechanical_Fault;, step_computed=, dynamic_computed=, step_sended=TLC_CONN=Connection*Operative_Level; TLC_SERVICE=TLC_services*Operative_Level+TLC_revoke*10;   CYBER_FAULT=Cyber_Fault*Operative_Level; MECH_FAULT=Mechanical_Fault;, id_entity=31, id_project=38, id_type=1, name_type=Optical_Wire, color=#99CCFF}
      mask prompts: Parameter1 "entity name"; Parameter2 "sampling time"; Parameter3 "project"; resources "input resources and state variables"; Parameter10 "Bring state variables to output"; codeupdate "update code from mask"
      mask help: This is a level-2 MATLAB file S-function which demonstrates CISIA entity
      mask DialogControl Container1 Prompt: All parameters
      mask Display: image('Icons/Optical_Wire.png')
  Wire_11 (36) : M-S-Function  FunctionName=cisia_msfun  Parameters=Parameter1, Parameter2, Parameter3, resources, Parameter10, codeupdate, step_received, step_computed, dynamic_computed, step_sended, id_entity, id_project, id_type, name_type, color  mask(S-function:msfcn_unit_delay){Parameter1='Wire_11', Parameter2=1, Parameter3='ORO', resources=*** INPUT RESOURCES *** NUM_INPUTS 4 TLC_CONN (20) TLC_SERVICE (20) CYBER_FAULT (10) MECH_FAULT (1)  *** STATE VARIABLES *** NUM_VARIABLES 11 Operative_Level(NUMERIC)(1)(1) TLC_services(NUMERIC_ARRAY)(20)(0  0  0  0  0  0  0  0  0  0  0  0  0  0  0  0  0  0  0  0) Connection(NUMERIC_ARRAY)(20)(0  0  0  0  0  0  0  0  0  0  0  0  0  0  0  0  0  0  0  0) Dos_attack(NUMERIC)(1)(0) MITM_attack(NUMERIC)(1)(0) Virus_Attack(NUMERIC)(1)(0) Port_Scan_Attack(NUMERIC)(1)(0) Cyber_Fault(NUMERIC_ARRAY)(10)(0  0  0  0  0  0  0  0  0  0) Mechanical_Fault(NUMERIC)(1)(0) Conn_Fault(NUMERIC)(1)(0) TLC_revoke(NUMERIC_ARRAY)(20)(0  0  0  0  0  0  0  0  0  0  0  0  0  0  0  0  0  0  0  0)  *** OUTPUT RESOURCES *** NUM_OUTPUTS 4 TLC_CONN (20) TLC_SERVICE (20) CYBER_FAULT (10) MECH_FAULT (1), Parameter10=off, codeupdate=off, step_received=Connection=max(Connection_init,TLC_CONN); TLC_services=max(TLC_services_init,TLC_SERVICE); TLC_services=mod(TLC_services,10); TLC_revoke=floor(TLC_SERVICE/10);  Cyber_Fault=CYBER_FAULT;  Mechanical_Fault=max([Mechanical_Fault MECH_FAULT Mechanical_Fault_init]);  %TLC_services=TLC_services.*(1-TLC_revoke);  Operative_Level=1-Mechanical_Fault;, step_computed=, dynamic_computed=, step_sended=TLC_CONN=Connection*Operative_Level; TLC_SERVICE=TLC_services*Operative_Level+TLC_revoke*10;   CYBER_FAULT=Cyber_Fault*Operative_Level; MECH_FAULT=Mechanical_Fault;, id_entity=36, id_project=38, id_type=1, name_type=Optical_Wire, color=#99CCFF}
      mask prompts: Parameter1 "entity name"; Parameter2 "sampling time"; Parameter3 "project"; resources "input resources and state variables"; Parameter10 "Bring state variables to output"; codeupdate "update code from mask"
      mask help: This is a level-2 MATLAB file S-function which demonstrates CISIA entity
      mask DialogControl Container1 Prompt: All parameters
      mask Display: image('Icons/Optical_Wire.png')
  Wire_11b (37) : M-S-Function  FunctionName=cisia_msfun  Parameters=Parameter1, Parameter2, Parameter3, resources, Parameter10, codeupdate, step_received, step_computed, dynamic_computed, step_sended, id_entity, id_project, id_type, name_type, color  mask(S-function:msfcn_unit_delay){Parameter1='Wire_11b', Parameter2=1, Parameter3='ORO', resources=*** INPUT RESOURCES *** NUM_INPUTS 4 TLC_CONN (20) TLC_SERVICE (20) CYBER_FAULT (10) MECH_FAULT (1)  *** STATE VARIABLES *** NUM_VARIABLES 11 Operative_Level(NUMERIC)(1)(1) TLC_services(NUMERIC_ARRAY)(20)(0  0  0  0  0  0  0  0  0  0  0  0  0  0  0  0  0  0  0  0) Connection(NUMERIC_ARRAY)(20)(0  0  0  0  0  0  0  0  0  0  0  0  0  0  0  0  0  0  0  0) Dos_attack(NUMERIC)(1)(0) MITM_attack(NUMERIC)(1)(0) Virus_Attack(NUMERIC)(1)(0) Port_Scan_Attack(NUMERIC)(1)(0) Cyber_Fault(NUMERIC_ARRAY)(10)(0  0  0  0  0  0  0  0  0  0) Mechanical_Fault(NUMERIC)(1)(0) Conn_Fault(NUMERIC)(1)(0) TLC_revoke(NUMERIC_ARRAY)(20)(0  0  0  0  0  0  0  0  0  0  0  0  0  0  0  0  0  0  0  0)  *** OUTPUT RESOURCES *** NUM_OUTPUTS 4 TLC_CONN (20) TLC_SERVICE (20) CYBER_FAULT (10) MECH_FAULT (1), Parameter10=off, codeupdate=off, step_received=Connection=max(Connection_init,TLC_CONN); TLC_services=max(TLC_services_init,TLC_SERVICE); TLC_services=mod(TLC_services,10); TLC_revoke=floor(TLC_SERVICE/10);  Cyber_Fault=CYBER_FAULT;  Mechanical_Fault=max([Mechanical_Fault MECH_FAULT Mechanical_Fault_init]);  %TLC_services=TLC_services.*(1-TLC_revoke);  Operative_Level=1-Mechanical_Fault;, step_computed=, dynamic_computed=, step_sended=TLC_CONN=Connection*Operative_Level; TLC_SERVICE=TLC_services*Operative_Level+TLC_revoke*10;   CYBER_FAULT=Cyber_Fault*Operative_Level; MECH_FAULT=Mechanical_Fault;, id_entity=37, id_project=38, id_type=1, name_type=Optical_Wire, color=#99CCFF}
      mask prompts: Parameter1 "entity name"; Parameter2 "sampling time"; Parameter3 "project"; resources "input resources and state variables"; Parameter10 "Bring state variables to output"; codeupdate "update code from mask"
      mask help: This is a level-2 MATLAB file S-function which demonstrates CISIA entity
      mask DialogControl Container1 Prompt: All parameters
      mask Display: image('Icons/Optical_Wire.png')
  Wire_12 (38) : M-S-Function  FunctionName=cisia_msfun  Parameters=Parameter1, Parameter2, Parameter3, resources, Parameter10, codeupdate, step_received, step_computed, dynamic_computed, step_sended, id_entity, id_project, id_type, name_type, color  mask(S-function:msfcn_unit_delay){Parameter1='Wire_12', Parameter2=1, Parameter3='ORO', resources=*** INPUT RESOURCES *** NUM_INPUTS 4 TLC_CONN (20) TLC_SERVICE (20) CYBER_FAULT (10) MECH_FAULT (1)  *** STATE VARIABLES *** NUM_VARIABLES 11 Operative_Level(NUMERIC)(1)(1) TLC_services(NUMERIC_ARRAY)(20)(0  0  0  0  0  0  0  0  0  0  0  0  0  0  0  0  0  0  0  0) Connection(NUMERIC_ARRAY)(20)(0  0  0  0  0  0  0  0  0  0  0  0  0  0  0  0  0  0  0  0) Dos_attack(NUMERIC)(1)(0) MITM_attack(NUMERIC)(1)(0) Virus_Attack(NUMERIC)(1)(0) Port_Scan_Attack(NUMERIC)(1)(0) Cyber_Fault(NUMERIC_ARRAY)(10)(0  0  0  0  0  0  0  0  0  0) Mechanical_Fault(NUMERIC)(1)(0) Conn_Fault(NUMERIC)(1)(0) TLC_revoke(NUMERIC_ARRAY)(20)(0  0  0  0  0  0  0  0  0  0  0  0  0  0  0  0  0  0  0  0)  *** OUTPUT RESOURCES *** NUM_OUTPUTS 4 TLC_CONN (20) TLC_SERVICE (20) CYBER_FAULT (10) MECH_FAULT (1), Parameter10=off, codeupdate=off, step_received=Connection=max(Connection_init,TLC_CONN); TLC_services=max(TLC_services_init,TLC_SERVICE); TLC_services=mod(TLC_services,10); TLC_revoke=floor(TLC_SERVICE/10);  Cyber_Fault=CYBER_FAULT;  Mechanical_Fault=max([Mechanical_Fault MECH_FAULT Mechanical_Fault_init]);  %TLC_services=TLC_services.*(1-TLC_revoke);  Operative_Level=1-Mechanical_Fault;, step_computed=, dynamic_computed=, step_sended=TLC_CONN=Connection*Operative_Level; TLC_SERVICE=TLC_services*Operative_Level+TLC_revoke*10;   CYBER_FAULT=Cyber_Fault*Operative_Level; MECH_FAULT=Mechanical_Fault;, id_entity=38, id_project=38, id_type=1, name_type=Optical_Wire, color=#99CCFF}
      mask prompts: Parameter1 "entity name"; Parameter2 "sampling time"; Parameter3 "project"; resources "input resources and state variables"; Parameter10 "Bring state variables to output"; codeupdate "update code from mask"
      mask help: This is a level-2 MATLAB file S-function which demonstrates CISIA entity
      mask DialogControl Container1 Prompt: All parameters
      mask Display: image('Icons/Optical_Wire.png')
  Wire_12b (39) : M-S-Function  FunctionName=cisia_msfun  Parameters=Parameter1, Parameter2, Parameter3, resources, Parameter10, codeupdate, step_received, step_computed, dynamic_computed, step_sended, id_entity, id_project, id_type, name_type, color  mask(S-function:msfcn_unit_delay){Parameter1='Wire_12b', Parameter2=1, Parameter3='ORO', resources=*** INPUT RESOURCES *** NUM_INPUTS 4 TLC_CONN (20) TLC_SERVICE (20) CYBER_FAULT (10) MECH_FAULT (1)  *** STATE VARIABLES *** NUM_VARIABLES 11 Operative_Level(NUMERIC)(1)(1) TLC_services(NUMERIC_ARRAY)(20)(0  0  0  0  0  0  0  0  0  0  0  0  0  0  0  0  0  0  0  0) Connection(NUMERIC_ARRAY)(20)(0  0  0  0  0  0  0  0  0  0  0  0  0  0  0  0  0  0  0  0) Dos_attack(NUMERIC)(1)(0) MITM_attack(NUMERIC)(1)(0) Virus_Attack(NUMERIC)(1)(0) Port_Scan_Attack(NUMERIC)(1)(0) Cyber_Fault(NUMERIC_ARRAY)(10)(0  0  0  0  0  0  0  0  0  0) Mechanical_Fault(NUMERIC)(1)(0) Conn_Fault(NUMERIC)(1)(0) TLC_revoke(NUMERIC_ARRAY)(20)(0  0  0  0  0  0  0  0  0  0  0  0  0  0  0  0  0  0  0  0)  *** OUTPUT RESOURCES *** NUM_OUTPUTS 4 TLC_CONN (20) TLC_SERVICE (20) CYBER_FAULT (10) MECH_FAULT (1), Parameter10=off, codeupdate=off, step_received=Connection=max(Connection_init,TLC_CONN); TLC_services=max(TLC_services_init,TLC_SERVICE); TLC_services=mod(TLC_services,10); TLC_revoke=floor(TLC_SERVICE/10);  Cyber_Fault=CYBER_FAULT;  Mechanical_Fault=max([Mechanical_Fault MECH_FAULT Mechanical_Fault_init]);  %TLC_services=TLC_services.*(1-TLC_revoke);  Operative_Level=1-Mechanical_Fault;, step_computed=, dynamic_computed=, step_sended=TLC_CONN=Connection*Operative_Level; TLC_SERVICE=TLC_services*Operative_Level+TLC_revoke*10;   CYBER_FAULT=Cyber_Fault*Operative_Level; MECH_FAULT=Mechanical_Fault;, id_entity=39, id_project=38, id_type=1, name_type=Optical_Wire, color=#99CCFF}
      mask prompts: Parameter1 "entity name"; Parameter2 "sampling time"; Parameter3 "project"; resources "input resources and state variables"; Parameter10 "Bring state variables to output"; codeupdate "update code from mask"
      mask help: This is a level-2 MATLAB file S-function which demonstrates CISIA entity
      mask DialogControl Container1 Prompt: All parameters
      mask Display: image('Icons/Optical_Wire.png')
  Wire_14 (42) : M-S-Function  FunctionName=cisia_msfun  Parameters=Parameter1, Parameter2, Parameter3, resources, Parameter10, codeupdate, step_received, step_computed, dynamic_computed, step_sended, id_entity, id_project, id_type, name_type, color  mask(S-function:msfcn_unit_delay){Parameter1='Wire_14', Parameter2=1, Parameter3='ORO', resources=*** INPUT RESOURCES *** NUM_INPUTS 4 TLC_CONN (20) TLC_SERVICE (20) CYBER_FAULT (10) MECH_FAULT (1)  *** STATE VARIABLES *** NUM_VARIABLES 11 Operative_Level(NUMERIC)(1)(1) TLC_services(NUMERIC_ARRAY)(20)(0  0  0  0  0  0  0  0  0  0  0  0  0  0  0  0  0  0  0  0) Connection(NUMERIC_ARRAY)(20)(0  0  0  0  0  0  0  0  0  0  0  0  0  0  0  0  0  0  0  0) Dos_attack(NUMERIC)(1)(0) MITM_attack(NUMERIC)(1)(0) Virus_Attack(NUMERIC)(1)(0) Port_Scan_Attack(NUMERIC)(1)(0) Cyber_Fault(NUMERIC_ARRAY)(10)(0  0  0  0  0  0  0  0  0  0) Mechanical_Fault(NUMERIC)(1)(0) Conn_Fault(NUMERIC)(1)(0) TLC_revoke(NUMERIC_ARRAY)(20)(0  0  0  0  0  0  0  0  0  0  0  0  0  0  0  0  0  0  0  0)  *** OUTPUT RESOURCES *** NUM_OUTPUTS 4 TLC_CONN (20) TLC_SERVICE (20) CYBER_FAULT (10) MECH_FAULT (1), Parameter10=off, codeupdate=off, step_received=Connection=max(Connection_init,TLC_CONN); TLC_services=max(TLC_services_init,TLC_SERVICE); TLC_services=mod(TLC_services,10); TLC_revoke=floor(TLC_SERVICE/10);  Cyber_Fault=CYBER_FAULT;  Mechanical_Fault=max([Mechanical_Fault MECH_FAULT Mechanical_Fault_init]);  %TLC_services=TLC_services.*(1-TLC_revoke);  Operative_Level=1-Mechanical_Fault;, step_computed=, dynamic_computed=, step_sended=TLC_CONN=Connection*Operative_Level; TLC_SERVICE=TLC_services*Operative_Level+TLC_revoke*10;   CYBER_FAULT=Cyber_Fault*Operative_Level; MECH_FAULT=Mechanical_Fault;, id_entity=42, id_project=38, id_type=1, name_type=Optical_Wire, color=#99CCFF}
      mask prompts: Parameter1 "entity name"; Parameter2 "sampling time"; Parameter3 "project"; resources "input resources and state variables"; Parameter10 "Bring state variables to output"; codeupdate "update code from mask"
      mask help: This is a level-2 MATLAB file S-function which demonstrates CISIA entity
      mask DialogControl Container1 Prompt: All parameters
      mask Display: image('Icons/Optical_Wire.png')
  Wire_14b (43) : M-S-Function  FunctionName=cisia_msfun  Parameters=Parameter1, Parameter2, Parameter3, resources, Parameter10, codeupdate, step_received, step_computed, dynamic_computed, step_sended, id_entity, id_project, id_type, name_type, color  mask(S-function:msfcn_unit_delay){Parameter1='Wire_14b', Parameter2=1, Parameter3='ORO', resources=*** INPUT RESOURCES *** NUM_INPUTS 4 TLC_CONN (20) TLC_SERVICE (20) CYBER_FAULT (10) MECH_FAULT (1)  *** STATE VARIABLES *** NUM_VARIABLES 11 Operative_Level(NUMERIC)(1)(1) TLC_services(NUMERIC_ARRAY)(20)(0  0  0  0  0  0  0  0  0  0  0  0  0  0  0  0  0  0  0  0) Connection(NUMERIC_ARRAY)(20)(0  0  0  0  0  0  0  0  0  0  0  0  0  0  0  0  0  0  0  0) Dos_attack(NUMERIC)(1)(0) MITM_attack(NUMERIC)(1)(0) Virus_Attack(NUMERIC)(1)(0) Port_Scan_Attack(NUMERIC)(1)(0) Cyber_Fault(NUMERIC_ARRAY)(10)(0  0  0  0  0  0  0  0  0  0) Mechanical_Fault(NUMERIC)(1)(0) Conn_Fault(NUMERIC)(1)(0) TLC_revoke(NUMERIC_ARRAY)(20)(0  0  0  0  0  0  0  0  0  0  0  0  0  0  0  0  0  0  0  0)  *** OUTPUT RESOURCES *** NUM_OUTPUTS 4 TLC_CONN (20) TLC_SERVICE (20) CYBER_FAULT (10) MECH_FAULT (1), Parameter10=off, codeupdate=off, step_received=Connection=max(Connection_init,TLC_CONN); TLC_services=max(TLC_services_init,TLC_SERVICE); TLC_services=mod(TLC_services,10); TLC_revoke=floor(TLC_SERVICE/10);  Cyber_Fault=CYBER_FAULT;  Mechanical_Fault=max([Mechanical_Fault MECH_FAULT Mechanical_Fault_init]);  %TLC_services=TLC_services.*(1-TLC_revoke);  Operative_Level=1-Mechanical_Fault;, step_computed=, dynamic_computed=, step_sended=TLC_CONN=Connection*Operative_Level; TLC_SERVICE=TLC_services*Operative_Level+TLC_revoke*10;   CYBER_FAULT=Cyber_Fault*Operative_Level; MECH_FAULT=Mechanical_Fault;, id_entity=43, id_project=38, id_type=1, name_type=Optical_Wire, color=#99CCFF}
      mask prompts: Parameter1 "entity name"; Parameter2 "sampling time"; Parameter3 "project"; resources "input resources and state variables"; Parameter10 "Bring state variables to output"; codeupdate "update code from mask"
      mask help: This is a level-2 MATLAB file S-function which demonstrates CISIA entity
      mask DialogControl Container1 Prompt: All parameters
      mask Display: image('Icons/Optical_Wire.png')
  Wire_15 (44) : M-S-Function  FunctionName=cisia_msfun  Parameters=Parameter1, Parameter2, Parameter3, resources, Parameter10, codeupdate, step_received, step_computed, dynamic_computed, step_sended, id_entity, id_project, id_type, name_type, color  mask(S-function:msfcn_unit_delay){Parameter1='Wire_15', Parameter2=1, Parameter3='ORO', resources=*** INPUT RESOURCES *** NUM_INPUTS 4 TLC_CONN (20) TLC_SERVICE (20) CYBER_FAULT (10) MECH_FAULT (1)  *** STATE VARIABLES *** NUM_VARIABLES 11 Operative_Level(NUMERIC)(1)(1) TLC_services(NUMERIC_ARRAY)(20)(0  0  0  0  0  0  0  0  0  0  0  0  0  0  0  0  0  0  0  0) Connection(NUMERIC_ARRAY)(20)(0  0  0  0  0  0  0  0  0  0  0  0  0  0  0  0  0  0  0  0) Dos_attack(NUMERIC)(1)(0) MITM_attack(NUMERIC)(1)(0) Virus_Attack(NUMERIC)(1)(0) Port_Scan_Attack(NUMERIC)(1)(0) Cyber_Fault(NUMERIC_ARRAY)(10)(0  0  0  0  0  0  0  0  0  0) Mechanical_Fault(NUMERIC)(1)(0) Conn_Fault(NUMERIC)(1)(0) TLC_revoke(NUMERIC_ARRAY)(20)(0  0  0  0  0  0  0  0  0  0  0  0  0  0  0  0  0  0  0  0)  *** OUTPUT RESOURCES *** NUM_OUTPUTS 4 TLC_CONN (20) TLC_SERVICE (20) CYBER_FAULT (10) MECH_FAULT (1), Parameter10=off, codeupdate=off, step_received=Connection=max(Connection_init,TLC_CONN); TLC_services=max(TLC_services_init,TLC_SERVICE); TLC_services=mod(TLC_services,10); TLC_revoke=floor(TLC_SERVICE/10);  Cyber_Fault=CYBER_FAULT;  Mechanical_Fault=max([Mechanical_Fault MECH_FAULT Mechanical_Fault_init]);  %TLC_services=TLC_services.*(1-TLC_revoke);  Operative_Level=1-Mechanical_Fault;, step_computed=, dynamic_computed=, step_sended=TLC_CONN=Connection*Operative_Level; TLC_SERVICE=TLC_services*Operative_Level+TLC_revoke*10;   CYBER_FAULT=Cyber_Fault*Operative_Level; MECH_FAULT=Mechanical_Fault;, id_entity=44, id_project=38, id_type=1, name_type=Optical_Wire, color=#99CCFF}
      mask prompts: Parameter1 "entity name"; Parameter2 "sampling time"; Parameter3 "project"; resources "input resources and state variables"; Parameter10 "Bring state variables to output"; codeupdate "update code from mask"
      mask help: This is a level-2 MATLAB file S-function which demonstrates CISIA entity
      mask DialogControl Container1 Prompt: All parameters
      mask Display: image('Icons/Optical_Wire.png')
  Wire_15a (49) : M-S-Function  FunctionName=cisia_msfun  Parameters=Parameter1, Parameter2, Parameter3, resources, Parameter10, codeupdate, step_received, step_computed, dynamic_computed, step_sended, id_entity, id_project, id_type, name_type, color  mask(S-function:msfcn_unit_delay){Parameter1='Wire_15a', Parameter2=1, Parameter3='ORO', resources=*** INPUT RESOURCES *** NUM_INPUTS 4 TLC_CONN (20) TLC_SERVICE (20) CYBER_FAULT (10) MECH_FAULT (1)  *** STATE VARIABLES *** NUM_VARIABLES 11 Operative_Level(NUMERIC)(1)(1) TLC_services(NUMERIC_ARRAY)(20)(0  0  0  0  0  0  0  0  0  0  0  0  0  0  0  0  0  0  0  0) Connection(NUMERIC_ARRAY)(20)(0  0  0  0  0  0  0  0  0  0  0  0  0  0  0  0  0  0  0  0) Dos_attack(NUMERIC)(1)(0) MITM_attack(NUMERIC)(1)(0) Virus_Attack(NUMERIC)(1)(0) Port_Scan_Attack(NUMERIC)(1)(0) Cyber_Fault(NUMERIC_ARRAY)(10)(0  0  0  0  0  0  0  0  0  0) Mechanical_Fault(NUMERIC)(1)(0) Conn_Fault(NUMERIC)(1)(0) TLC_revoke(NUMERIC_ARRAY)(20)(0  0  0  0  0  0  0  0  0  0  0  0  0  0  0  0  0  0  0  0)  *** OUTPUT RESOURCES *** NUM_OUTPUTS 4 TLC_CONN (20) TLC_SERVICE (20) CYBER_FAULT (10) MECH_FAULT (1), Parameter10=off, codeupdate=off, step_received=Connection=max(Connection_init,TLC_CONN); TLC_services=max(TLC_services_init,TLC_SERVICE); TLC_services=mod(TLC_services,10); TLC_revoke=floor(TLC_SERVICE/10);  Cyber_Fault=CYBER_FAULT;  Mechanical_Fault=max([Mechanical_Fault MECH_FAULT Mechanical_Fault_init]);  %TLC_services=TLC_services.*(1-TLC_revoke);  Operative_Level=1-Mechanical_Fault;, step_computed=, dynamic_computed=, step_sended=TLC_CONN=Connection*Operative_Level; TLC_SERVICE=TLC_services*Operative_Level+TLC_revoke*10;   CYBER_FAULT=Cyber_Fault*Operative_Level; MECH_FAULT=Mechanical_Fault;, id_entity=49, id_project=38, id_type=1, name_type=Optical_Wire, color=#99CCFF}
      mask prompts: Parameter1 "entity name"; Parameter2 "sampling time"; Parameter3 "project"; resources "input resources and state variables"; Parameter10 "Bring state variables to output"; codeupdate "update code from mask"
      mask help: This is a level-2 MATLAB file S-function which demonstrates CISIA entity
      mask DialogControl Container1 Prompt: All parameters
      mask Display: image('Icons/Optical_Wire.png')
  Wire_16 (45) : M-S-Function  FunctionName=cisia_msfun  Parameters=Parameter1, Parameter2, Parameter3, resources, Parameter10, codeupdate, step_received, step_computed, dynamic_computed, step_sended, id_entity, id_project, id_type, name_type, color  mask(S-function:msfcn_unit_delay){Parameter1='Wire_16', Parameter2=1, Parameter3='ORO', resources=*** INPUT RESOURCES *** NUM_INPUTS 4 TLC_CONN (20) TLC_SERVICE (20) CYBER_FAULT (10) MECH_FAULT (1)  *** STATE VARIABLES *** NUM_VARIABLES 11 Operative_Level(NUMERIC)(1)(1) TLC_services(NUMERIC_ARRAY)(20)(0  0  0  0  0  0  0  0  0  0  0  0  0  0  0  0  0  0  0  0) Connection(NUMERIC_ARRAY)(20)(0  0  0  0  0  0  0  0  0  0  0  0  0  0  0  0  0  0  0  0) Dos_attack(NUMERIC)(1)(0) MITM_attack(NUMERIC)(1)(0) Virus_Attack(NUMERIC)(1)(0) Port_Scan_Attack(NUMERIC)(1)(0) Cyber_Fault(NUMERIC_ARRAY)(10)(0  0  0  0  0  0  0  0  0  0) Mechanical_Fault(NUMERIC)(1)(0) Conn_Fault(NUMERIC)(1)(0) TLC_revoke(NUMERIC_ARRAY)(20)(0  0  0  0  0  0  0  0  0  0  0  0  0  0  0  0  0  0  0  0)  *** OUTPUT RESOURCES *** NUM_OUTPUTS 4 TLC_CONN (20) TLC_SERVICE (20) CYBER_FAULT (10) MECH_FAULT (1), Parameter10=off, codeupdate=off, step_received=Connection=max(Connection_init,TLC_CONN); TLC_services=max(TLC_services_init,TLC_SERVICE); TLC_services=mod(TLC_services,10); TLC_revoke=floor(TLC_SERVICE/10);  Cyber_Fault=CYBER_FAULT;  Mechanical_Fault=max([Mechanical_Fault MECH_FAULT Mechanical_Fault_init]);  %TLC_services=TLC_services.*(1-TLC_revoke);  Operative_Level=1-Mechanical_Fault;, step_computed=, dynamic_computed=, step_sended=TLC_CONN=Connection*Operative_Level; TLC_SERVICE=TLC_services*Operative_Level+TLC_revoke*10;   CYBER_FAULT=Cyber_Fault*Operative_Level; MECH_FAULT=Mechanical_Fault;, id_entity=45, id_project=38, id_type=1, name_type=Optical_Wire, color=#99CCFF}
      mask prompts: Parameter1 "entity name"; Parameter2 "sampling time"; Parameter3 "project"; resources "input resources and state variables"; Parameter10 "Bring state variables to output"; codeupdate "update code from mask"
      mask help: This is a level-2 MATLAB file S-function which demonstrates CISIA entity
      mask DialogControl Container1 Prompt: All parameters
      mask Display: image('Icons/Optical_Wire.png')
